simulink model "v2012_DynStab"  (Simulink 7.6)
settings: Solver=ode45  StartTime=0.0  StopTime=10.0  RelTol=1e-3
libraries: fm_lib x1
(part 1 of 4)
settings Model: Creator=davidusb  LastModifiedBy=davidusb

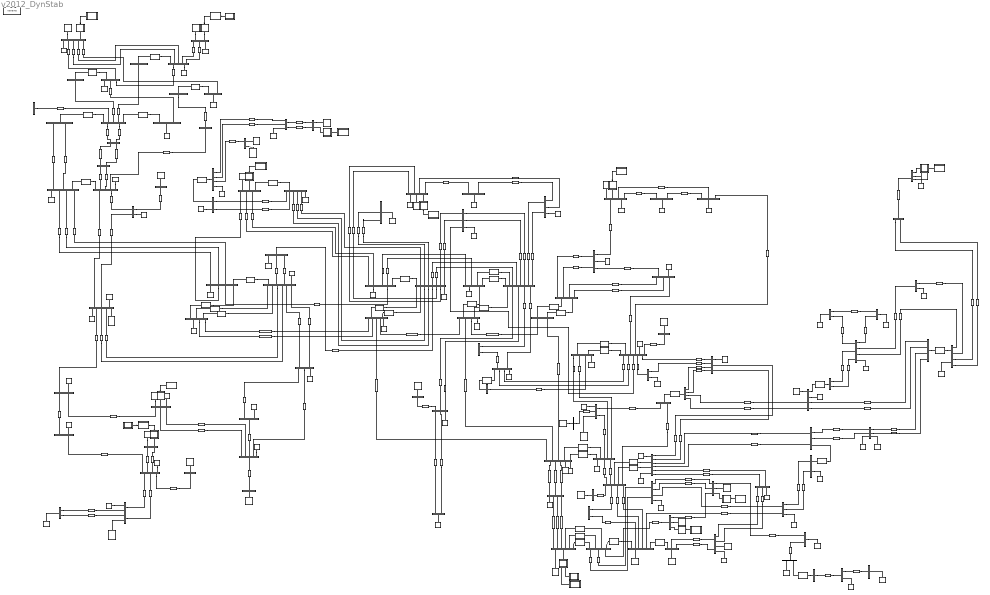
== system v2012_DynStab ==
  note: Hacia Empresas
      | Mixtas PDVSA
  note: REACTOR
      | 3x300
  note: REACTOR
      | 4x300
  note: COMP
      | ESTATICO
  note: REACTOR
      | 2x50
  note: Guri 400 kV
  note: Macagua I y III
  note: Caruachi
  note: Macagua II
  note: S/E San Geronimo 765kV
  note: S/E Malena 765kV
  note: S/E Guri 765kV
  note: Ciudad
      | Guayana
  note: Guri 230 kV
  note: Droop = ~0 ==> isochronous mode
  note: (AT adicional 150MVA 2012)
  note: 2x100MVAr
      | SHUNT CAP
  note: Puerto La Cruz
  note: Caracas
  note: Maracay
  note: S/E Sur 765kV
  note: REACTOR
      | 2x100
  note: (2da linea 2012)
  note: Valencia
  note: S/E La Horqueta 765kV
  note: S/E La Arenosa 765kV
  note: LIBRE
  note: Elaborado por: Ing. David Hernández Torres, PhD
      |
      | VERSION: 20 de Noviembre de 2012 (Simplificada, niveles de tensión: 765, 400 y 230 kV)
      | (Solo se considera una pequeña parte de la red oriental en 115kV)
      | Modelo dinámico para estudios de estabilidad
      |
      | Fuentes:
      | Elaborado siguiendo diagrama unifilar actualizado hasta el 2003 (OPSIS) y las actualizaciones
      | del sistema descritas en el Anuario Estadístico del MPPEE hasta el año 2010 y en los
      | informe anuales OPSIS 2005-2008. Finalmente el modelo 2012 se obtiene luego de actualización
      | del modelo 2010 bajo las premisas descritas en los archivos pronostico_demanda_electrica.xls y
      | Datos SEN.xls
      |
      | (Es necesaria la instalación del toolbox PSAT, el esquema se elaboró con Simulink
      | y la version 7.11 R2010b de Matlab, se puede ejecutar el archivo de datos .m desde Octave y la
      | version de PSAT correspondiente)
  note: SISTEMA ELECTRICO NACIONAL
  note: COMP
      | ESTATICO
  note: REACTOR
      | 2x50
  note: REACTOR
      | 1x300
  note: REACTOR
      | 2x25
  note: Cumana
  note: REACTOR
      | 1x50
  note: Isla de Margarita
  note: REACTOR
      | 2x25
  note: Brasil
  note: REACTOR
      | 2x50
  note: TAP=1.1
  note: Termozulia
      | Rafael Urdaneta
  note: CAPACITOR
      | 1x108
  note: REACTOR
      | 1x50
  note: REACTOR
      | 4x50
  note: SERIES
      | CAPACITOR
      | COMP
      | 3x50 OHM
  note: Maracaibo
  note: HACIA COLOMBIA
  note: REACTOR
      | 1x300
  note: REACTOR
      | 4x50
  note: LIBRE
  note: LIBRE
  note: S/E Yaracuy 765kV
  note: Barquisimeto
  note: Merida
  note: San Cristobal
  note: Colombia
  note: REACTOR
      | 2x20
  note: Peninsula de Paraguaná
  note: (2da linea 2012)
  AVR1 : Subsystem  Tag=PSATblock  Description=Controls  mask(Exc){p2q=2, p3q=inf, p4q=0, p5q=200, p6q=0.02, p7q=0.01, p8q=1.0, p9q=1, p10q=0.7, p11q=0.001, p12_13q=[0.0006  0.9], in=0}
      mask prompts: p2q "Automatic Voltage Regulator Type"; p3q "Maximum Regulator Voltage [p.u.]"; p4q "Minimum Regulator Voltage [p.u.]"; p5q "Amplifier Gain Ka [p.u./p.u.]"; p6q "Amplifier Time Constant Ta [s]"; p7q "Stabilizer Gain Kf [p.u./p.u.]"; p8q "Stabilizer Time Tf [s]"; p9q "Integral deviation Ke [p.u./p.u.]"; p10q "Time Constant of the Field Circuit Td [s]"; p11q "Time Delay of the Measurement System Tr [s]"; p12_13q "Coefficient of the Ceiling Function (A B)"; in "Number of input signals"
      mask help: This block defines an Automatic Voltage Regulator.
      mask init:
      | fm_inout
      | [x,y] = fm_draw('R');
      mask Help:
      | This block defines an Automatic Voltage Regulator.
      | There are three kind of regulators:
      | 
      | Type 1:
      | 
      |      IEEE Model 1
      | 
      | Type 2:
      | 
      |      IEEE Model 2
      | 
      | Type 3:
      | 
      |      IEEE Model 3
      mask StyleString: popup(1|2|3),edit,edit,edit,edit,edit,edit,edit,edit,edit,edit,popup(0|1|2|3)
      mask CallbackString: fm_block|||||||||||
      mask Display:
      | plot([-1.8 4.1 4.1 -1.8 -1.8],[-1.5 -1.5 1.5 1.5 -1.5])
      | color('red')
      | plot([-1.3 -0.5],[-1 1],[-0.5 0.3],[1 -1],[-0.9 -0.1],[0.0 0.0])
      | plot(2.8+1.3*x,2*y,1.5+[-1.3 -0.5],[1 -1],1.5+[-0.5 0.3],[-1 1])
  AVR10 : Subsystem  Tag=PSATblock  Description=Controls  mask(Exc){p2q=2, p3q=7.3, p4q=-7.3, p5q=400, p6q=0.02, p7q=0.03, p8q=1.0, p9q=1, p10q=0.253, p11q=0.001, p12_13q=[0.0006  0.9], in=0}
      mask prompts: p2q "Automatic Voltage Regulator Type"; p3q "Maximum Regulator Voltage [p.u.]"; p4q "Minimum Regulator Voltage [p.u.]"; p5q "Amplifier Gain Ka [p.u./p.u.]"; p6q "Amplifier Time Constant Ta [s]"; p7q "Stabilizer Gain Kf [p.u./p.u.]"; p8q "Stabilizer Time Tf [s]"; p9q "Integral deviation Ke [p.u./p.u.]"; p10q "Time Constant of the Field Circuit Td [s]"; p11q "Time Delay of the Measurement System Tr [s]"; p12_13q "Coefficient of the Ceiling Function (A B)"; in "Number of input signals"
      mask help: This block defines an Automatic Voltage Regulator.
      mask init:
      | fm_inout
      | [x,y] = fm_draw('R');
      mask Help:
      | This block defines an Automatic Voltage Regulator.
      | There are three kind of regulators:
      | 
      | Type 1:
      | 
      |      IEEE Model 1
      | 
      | Type 2:
      | 
      |      IEEE Model 2
      | 
      | Type 3:
      | 
      |      IEEE Model 3
      mask StyleString: popup(1|2|3),edit,edit,edit,edit,edit,edit,edit,edit,edit,edit,popup(0|1|2|3)
      mask CallbackString: fm_block|||||||||||
      mask Display:
      | plot([-1.8 4.1 4.1 -1.8 -1.8],[-1.5 -1.5 1.5 1.5 -1.5])
      | color('red')
      | plot([-1.3 -0.5],[-1 1],[-0.5 0.3],[1 -1],[-0.9 -0.1],[0.0 0.0])
      | plot(2.8+1.3*x,2*y,1.5+[-1.3 -0.5],[1 -1],1.5+[-0.5 0.3],[-1 1])
  AVR11 : Subsystem  Tag=PSATblock  Description=Controls  mask(Exc){p2q=2, p3q=7.3, p4q=-7.3, p5q=400, p6q=0.02, p7q=0.03, p8q=1.0, p9q=1, p10q=0.253, p11q=0.001, p12_13q=[0.0006  0.9], in=0}
      mask prompts: p2q "Automatic Voltage Regulator Type"; p3q "Maximum Regulator Voltage [p.u.]"; p4q "Minimum Regulator Voltage [p.u.]"; p5q "Amplifier Gain Ka [p.u./p.u.]"; p6q "Amplifier Time Constant Ta [s]"; p7q "Stabilizer Gain Kf [p.u./p.u.]"; p8q "Stabilizer Time Tf [s]"; p9q "Integral deviation Ke [p.u./p.u.]"; p10q "Time Constant of the Field Circuit Td [s]"; p11q "Time Delay of the Measurement System Tr [s]"; p12_13q "Coefficient of the Ceiling Function (A B)"; in "Number of input signals"
      mask help: This block defines an Automatic Voltage Regulator.
      mask init:
      | fm_inout
      | [x,y] = fm_draw('R');
      mask Help:
      | This block defines an Automatic Voltage Regulator.
      | There are three kind of regulators:
      | 
      | Type 1:
      | 
      |      IEEE Model 1
      | 
      | Type 2:
      | 
      |      IEEE Model 2
      | 
      | Type 3:
      | 
      |      IEEE Model 3
      mask StyleString: popup(1|2|3),edit,edit,edit,edit,edit,edit,edit,edit,edit,edit,popup(0|1|2|3)
      mask CallbackString: fm_block|||||||||||
      mask Display:
      | plot([-1.8 4.1 4.1 -1.8 -1.8],[-1.5 -1.5 1.5 1.5 -1.5])
      | color('red')
      | plot([-1.3 -0.5],[-1 1],[-0.5 0.3],[1 -1],[-0.9 -0.1],[0.0 0.0])
      | plot(2.8+1.3*x,2*y,1.5+[-1.3 -0.5],[1 -1],1.5+[-0.5 0.3],[-1 1])
  AVR12 : Subsystem  Tag=PSATblock  Description=Controls  mask(Exc){p2q=2, p3q=50, p4q=-7.3, p5q=400, p6q=0.02, p7q=0.03, p8q=1.0, p9q=1, p10q=0.253, p11q=0.001, p12_13q=[0.0006  0.9], in=0}
      mask prompts: p2q "Automatic Voltage Regulator Type"; p3q "Maximum Regulator Voltage [p.u.]"; p4q "Minimum Regulator Voltage [p.u.]"; p5q "Amplifier Gain Ka [p.u./p.u.]"; p6q "Amplifier Time Constant Ta [s]"; p7q "Stabilizer Gain Kf [p.u./p.u.]"; p8q "Stabilizer Time Tf [s]"; p9q "Integral deviation Ke [p.u./p.u.]"; p10q "Time Constant of the Field Circuit Td [s]"; p11q "Time Delay of the Measurement System Tr [s]"; p12_13q "Coefficient of the Ceiling Function (A B)"; in "Number of input signals"
      mask help: This block defines an Automatic Voltage Regulator.
      mask init:
      | fm_inout
      | [x,y] = fm_draw('R');
      mask Help:
      | This block defines an Automatic Voltage Regulator.
      | There are three kind of regulators:
      | 
      | Type 1:
      | 
      |      IEEE Model 1
      | 
      | Type 2:
      | 
      |      IEEE Model 2
      | 
      | Type 3:
      | 
      |      IEEE Model 3
      mask StyleString: popup(1|2|3),edit,edit,edit,edit,edit,edit,edit,edit,edit,edit,popup(0|1|2|3)
      mask CallbackString: fm_block|||||||||||
      mask Display:
      | plot([-1.8 4.1 4.1 -1.8 -1.8],[-1.5 -1.5 1.5 1.5 -1.5])
      | color('red')
      | plot([-1.3 -0.5],[-1 1],[-0.5 0.3],[1 -1],[-0.9 -0.1],[0.0 0.0])
      | plot(2.8+1.3*x,2*y,1.5+[-1.3 -0.5],[1 -1],1.5+[-0.5 0.3],[-1 1])
  AVR13 : Subsystem  Tag=PSATblock  Description=Controls  mask(Exc){p2q=2, p3q=50, p4q=-3.84, p5q=200, p6q=0.395, p7q=0.0635, p8q=1.0, p9q=1, p10q=0.001, p11q=0.001, p12_13q=[0.0006  0.9], in=0}
      mask prompts: p2q "Automatic Voltage Regulator Type"; p3q "Maximum Regulator Voltage [p.u.]"; p4q "Minimum Regulator Voltage [p.u.]"; p5q "Amplifier Gain Ka [p.u./p.u.]"; p6q "Amplifier Time Constant Ta [s]"; p7q "Stabilizer Gain Kf [p.u./p.u.]"; p8q "Stabilizer Time Tf [s]"; p9q "Integral deviation Ke [p.u./p.u.]"; p10q "Time Constant of the Field Circuit Td [s]"; p11q "Time Delay of the Measurement System Tr [s]"; p12_13q "Coefficient of the Ceiling Function (A B)"; in "Number of input signals"
      mask help: This block defines an Automatic Voltage Regulator.
      mask init:
      | fm_inout
      | [x,y] = fm_draw('R');
      mask Help:
      | This block defines an Automatic Voltage Regulator.
      | There are three kind of regulators:
      | 
      | Type 1:
      | 
      |      IEEE Model 1
      | 
      | Type 2:
      | 
      |      IEEE Model 2
      | 
      | Type 3:
      | 
      |      IEEE Model 3
      mask StyleString: popup(1|2|3),edit,edit,edit,edit,edit,edit,edit,edit,edit,edit,popup(0|1|2|3)
      mask CallbackString: fm_block|||||||||||
      mask Display:
      | plot([-1.8 4.1 4.1 -1.8 -1.8],[-1.5 -1.5 1.5 1.5 -1.5])
      | color('red')
      | plot([-1.3 -0.5],[-1 1],[-0.5 0.3],[1 -1],[-0.9 -0.1],[0.0 0.0])
      | plot(2.8+1.3*x,2*y,1.5+[-1.3 -0.5],[1 -1],1.5+[-0.5 0.3],[-1 1])
  AVR2 : Subsystem  Tag=PSATblock  Description=Controls  mask(Exc){p2q=2, p3q=7.3, p4q=-7.3, p5q=400, p6q=0.02, p7q=0.03, p8q=1.0, p9q=1, p10q=0.253, p11q=0.001, p12_13q=[0.0006  0.9], in=0}
      mask prompts: p2q "Automatic Voltage Regulator Type"; p3q "Maximum Regulator Voltage [p.u.]"; p4q "Minimum Regulator Voltage [p.u.]"; p5q "Amplifier Gain Ka [p.u./p.u.]"; p6q "Amplifier Time Constant Ta [s]"; p7q "Stabilizer Gain Kf [p.u./p.u.]"; p8q "Stabilizer Time Tf [s]"; p9q "Integral deviation Ke [p.u./p.u.]"; p10q "Time Constant of the Field Circuit Td [s]"; p11q "Time Delay of the Measurement System Tr [s]"; p12_13q "Coefficient of the Ceiling Function (A B)"; in "Number of input signals"
      mask help: This block defines an Automatic Voltage Regulator.
      mask init:
      | fm_inout
      | [x,y] = fm_draw('R');
      mask Help:
      | This block defines an Automatic Voltage Regulator.
      | There are three kind of regulators:
      | 
      | Type 1:
      | 
      |      IEEE Model 1
      | 
      | Type 2:
      | 
      |      IEEE Model 2
      | 
      | Type 3:
      | 
      |      IEEE Model 3
      mask StyleString: popup(1|2|3),edit,edit,edit,edit,edit,edit,edit,edit,edit,edit,popup(0|1|2|3)
      mask CallbackString: fm_block|||||||||||
      mask Display:
      | plot([-1.8 4.1 4.1 -1.8 -1.8],[-1.5 -1.5 1.5 1.5 -1.5])
      | color('red')
      | plot([-1.3 -0.5],[-1 1],[-0.5 0.3],[1 -1],[-0.9 -0.1],[0.0 0.0])
      | plot(2.8+1.3*x,2*y,1.5+[-1.3 -0.5],[1 -1],1.5+[-0.5 0.3],[-1 1])
  AVR3 : Subsystem  Tag=PSATblock  Description=Controls  mask(Exc){p2q=2, p3q=1, p4q=-1, p5q=50, p6q=0.06, p7q=0.07, p8q=1.0, p9q=-0.0393, p10q=0.44, p11q=0.001, p12_13q=[0.0006  0.9], in=1}
      mask prompts: p2q "Automatic Voltage Regulator Type"; p3q "Maximum Regulator Voltage [p.u.]"; p4q "Minimum Regulator Voltage [p.u.]"; p5q "Amplifier Gain Ka [p.u./p.u.]"; p6q "Amplifier Time Constant Ta [s]"; p7q "Stabilizer Gain Kf [p.u./p.u.]"; p8q "Stabilizer Time Tf [s]"; p9q "Integral deviation Ke [p.u./p.u.]"; p10q "Time Constant of the Field Circuit Td [s]"; p11q "Time Delay of the Measurement System Tr [s]"; p12_13q "Coefficient of the Ceiling Function (A B)"; in "Number of input signals"
      mask help: This block defines an Automatic Voltage Regulator.
      mask init:
      | fm_inout
      | [x,y] = fm_draw('R');
      mask Help:
      | This block defines an Automatic Voltage Regulator.
      | There are three kind of regulators:
      | 
      | Type 1:
      | 
      |      IEEE Model 1
      | 
      | Type 2:
      | 
      |      IEEE Model 2
      | 
      | Type 3:
      | 
      |      IEEE Model 3
      mask StyleString: popup(1|2|3),edit,edit,edit,edit,edit,edit,edit,edit,edit,edit,popup(0|1|2|3)
      mask CallbackString: fm_block|||||||||||
      mask Display:
      | plot([-1.8 4.1 4.1 -1.8 -1.8],[-1.5 -1.5 1.5 1.5 -1.5])
      | color('red')
      | plot([-1.3 -0.5],[-1 1],[-0.5 0.3],[1 -1],[-0.9 -0.1],[0.0 0.0])
      | plot(2.8+1.3*x,2*y,1.5+[-1.3 -0.5],[1 -1],1.5+[-0.5 0.3],[-1 1])
  AVR4 : Subsystem  Tag=PSATblock  Description=Controls  mask(Exc){p2q=2, p3q=10, p4q=-3.84, p5q=200, p6q=0.395, p7q=0.0635, p8q=1.0, p9q=1, p10q=0.001, p11q=0.001, p12_13q=[0.0006  0.9], in=0}
      mask prompts: p2q "Automatic Voltage Regulator Type"; p3q "Maximum Regulator Voltage [p.u.]"; p4q "Minimum Regulator Voltage [p.u.]"; p5q "Amplifier Gain Ka [p.u./p.u.]"; p6q "Amplifier Time Constant Ta [s]"; p7q "Stabilizer Gain Kf [p.u./p.u.]"; p8q "Stabilizer Time Tf [s]"; p9q "Integral deviation Ke [p.u./p.u.]"; p10q "Time Constant of the Field Circuit Td [s]"; p11q "Time Delay of the Measurement System Tr [s]"; p12_13q "Coefficient of the Ceiling Function (A B)"; in "Number of input signals"
      mask help: This block defines an Automatic Voltage Regulator.
      mask init:
      | fm_inout
      | [x,y] = fm_draw('R');
      mask Help:
      | This block defines an Automatic Voltage Regulator.
      | There are three kind of regulators:
      | 
      | Type 1:
      | 
      |      IEEE Model 1
      | 
      | Type 2:
      | 
      |      IEEE Model 2
      | 
      | Type 3:
      | 
      |      IEEE Model 3
      mask StyleString: popup(1|2|3),edit,edit,edit,edit,edit,edit,edit,edit,edit,edit,popup(0|1|2|3)
      mask CallbackString: fm_block|||||||||||
      mask Display:
      | plot([-1.8 4.1 4.1 -1.8 -1.8],[-1.5 -1.5 1.5 1.5 -1.5])
      | color('red')
      | plot([-1.3 -0.5],[-1 1],[-0.5 0.3],[1 -1],[-0.9 -0.1],[0.0 0.0])
      | plot(2.8+1.3*x,2*y,1.5+[-1.3 -0.5],[1 -1],1.5+[-0.5 0.3],[-1 1])
  AVR5 : Subsystem  Tag=PSATblock  Description=Controls  mask(Exc){p2q=2, p3q=10, p4q=-1, p5q=50, p6q=0.06, p7q=0.0648, p8q=1.0, p9q=-0.08, p10q=0.405, p11q=0.001, p12_13q=[0.0006  0.9], in=0}
      mask prompts: p2q "Automatic Voltage Regulator Type"; p3q "Maximum Regulator Voltage [p.u.]"; p4q "Minimum Regulator Voltage [p.u.]"; p5q "Amplifier Gain Ka [p.u./p.u.]"; p6q "Amplifier Time Constant Ta [s]"; p7q "Stabilizer Gain Kf [p.u./p.u.]"; p8q "Stabilizer Time Tf [s]"; p9q "Integral deviation Ke [p.u./p.u.]"; p10q "Time Constant of the Field Circuit Td [s]"; p11q "Time Delay of the Measurement System Tr [s]"; p12_13q "Coefficient of the Ceiling Function (A B)"; in "Number of input signals"
      mask help: This block defines an Automatic Voltage Regulator.
      mask init:
      | fm_inout
      | [x,y] = fm_draw('R');
      mask Help:
      | This block defines an Automatic Voltage Regulator.
      | There are three kind of regulators:
      | 
      | Type 1:
      | 
      |      IEEE Model 1
      | 
      | Type 2:
      | 
      |      IEEE Model 2
      | 
      | Type 3:
      | 
      |      IEEE Model 3
      mask StyleString: popup(1|2|3),edit,edit,edit,edit,edit,edit,edit,edit,edit,edit,popup(0|1|2|3)
      mask CallbackString: fm_block|||||||||||
      mask Display:
      | plot([-1.8 4.1 4.1 -1.8 -1.8],[-1.5 -1.5 1.5 1.5 -1.5])
      | color('red')
      | plot([-1.3 -0.5],[-1 1],[-0.5 0.3],[1 -1],[-0.9 -0.1],[0.0 0.0])
      | plot(2.8+1.3*x,2*y,1.5+[-1.3 -0.5],[1 -1],1.5+[-0.5 0.3],[-1 1])
  AVR6 : Subsystem  Tag=PSATblock  Description=Controls  mask(Exc){p2q=2, p3q=inf, p4q=-1, p5q=50, p6q=0.06, p7q=0.0648, p8q=1.0, p9q=-0.08, p10q=0.405, p11q=0.001, p12_13q=[0.0006  0.9], in=0}
      mask prompts: p2q "Automatic Voltage Regulator Type"; p3q "Maximum Regulator Voltage [p.u.]"; p4q "Minimum Regulator Voltage [p.u.]"; p5q "Amplifier Gain Ka [p.u./p.u.]"; p6q "Amplifier Time Constant Ta [s]"; p7q "Stabilizer Gain Kf [p.u./p.u.]"; p8q "Stabilizer Time Tf [s]"; p9q "Integral deviation Ke [p.u./p.u.]"; p10q "Time Constant of the Field Circuit Td [s]"; p11q "Time Delay of the Measurement System Tr [s]"; p12_13q "Coefficient of the Ceiling Function (A B)"; in "Number of input signals"
      mask help: This block defines an Automatic Voltage Regulator.
      mask init:
      | fm_inout
      | [x,y] = fm_draw('R');
      mask Help:
      | This block defines an Automatic Voltage Regulator.
      | There are three kind of regulators:
      | 
      | Type 1:
      | 
      |      IEEE Model 1
      | 
      | Type 2:
      | 
      |      IEEE Model 2
      | 
      | Type 3:
      | 
      |      IEEE Model 3
      mask StyleString: popup(1|2|3),edit,edit,edit,edit,edit,edit,edit,edit,edit,edit,popup(0|1|2|3)
      mask CallbackString: fm_block|||||||||||
      mask Display:
      | plot([-1.8 4.1 4.1 -1.8 -1.8],[-1.5 -1.5 1.5 1.5 -1.5])
      | color('red')
      | plot([-1.3 -0.5],[-1 1],[-0.5 0.3],[1 -1],[-0.9 -0.1],[0.0 0.0])
      | plot(2.8+1.3*x,2*y,1.5+[-1.3 -0.5],[1 -1],1.5+[-0.5 0.3],[-1 1])
  AVR7 : Subsystem  Tag=PSATblock  Description=Controls  mask(Exc){p2q=2, p3q=1, p4q=-1, p5q=50, p6q=0.06, p7q=0.0648, p8q=1.0, p9q=-0.08, p10q=0.405, p11q=0.001, p12_13q=[0.0006  0.9], in=0}
      mask prompts: p2q "Automatic Voltage Regulator Type"; p3q "Maximum Regulator Voltage [p.u.]"; p4q "Minimum Regulator Voltage [p.u.]"; p5q "Amplifier Gain Ka [p.u./p.u.]"; p6q "Amplifier Time Constant Ta [s]"; p7q "Stabilizer Gain Kf [p.u./p.u.]"; p8q "Stabilizer Time Tf [s]"; p9q "Integral deviation Ke [p.u./p.u.]"; p10q "Time Constant of the Field Circuit Td [s]"; p11q "Time Delay of the Measurement System Tr [s]"; p12_13q "Coefficient of the Ceiling Function (A B)"; in "Number of input signals"
      mask help: This block defines an Automatic Voltage Regulator.
      mask init:
      | fm_inout
      | [x,y] = fm_draw('R');
      mask Help:
      | This block defines an Automatic Voltage Regulator.
      | There are three kind of regulators:
      | 
      | Type 1:
      | 
      |      IEEE Model 1
      | 
      | Type 2:
      | 
      |      IEEE Model 2
      | 
      | Type 3:
      | 
      |      IEEE Model 3
      mask StyleString: popup(1|2|3),edit,edit,edit,edit,edit,edit,edit,edit,edit,edit,popup(0|1|2|3)
      mask CallbackString: fm_block|||||||||||
      mask Display:
      | plot([-1.8 4.1 4.1 -1.8 -1.8],[-1.5 -1.5 1.5 1.5 -1.5])
      | color('red')
      | plot([-1.3 -0.5],[-1 1],[-0.5 0.3],[1 -1],[-0.9 -0.1],[0.0 0.0])
      | plot(2.8+1.3*x,2*y,1.5+[-1.3 -0.5],[1 -1],1.5+[-0.5 0.3],[-1 1])
  AVR8 : Subsystem  Tag=PSATblock  Description=Controls  mask(Exc){p2q=2, p3q=1, p4q=-1, p5q=50, p6q=0.06, p7q=0.0648, p8q=1.0, p9q=-0.08, p10q=0.405, p11q=0.001, p12_13q=[0.0006  0.9], in=1}
      mask prompts: p2q "Automatic Voltage Regulator Type"; p3q "Maximum Regulator Voltage [p.u.]"; p4q "Minimum Regulator Voltage [p.u.]"; p5q "Amplifier Gain Ka [p.u./p.u.]"; p6q "Amplifier Time Constant Ta [s]"; p7q "Stabilizer Gain Kf [p.u./p.u.]"; p8q "Stabilizer Time Tf [s]"; p9q "Integral deviation Ke [p.u./p.u.]"; p10q "Time Constant of the Field Circuit Td [s]"; p11q "Time Delay of the Measurement System Tr [s]"; p12_13q "Coefficient of the Ceiling Function (A B)"; in "Number of input signals"
      mask help: This block defines an Automatic Voltage Regulator.
      mask init:
      | fm_inout
      | [x,y] = fm_draw('R');
      mask Help:
      | This block defines an Automatic Voltage Regulator.
      | There are three kind of regulators:
      | 
      | Type 1:
      | 
      |      IEEE Model 1
      | 
      | Type 2:
      | 
      |      IEEE Model 2
      | 
      | Type 3:
      | 
      |      IEEE Model 3
      mask StyleString: popup(1|2|3),edit,edit,edit,edit,edit,edit,edit,edit,edit,edit,popup(0|1|2|3)
      mask CallbackString: fm_block|||||||||||
      mask Display:
      | plot([-1.8 4.1 4.1 -1.8 -1.8],[-1.5 -1.5 1.5 1.5 -1.5])
      | color('red')
      | plot([-1.3 -0.5],[-1 1],[-0.5 0.3],[1 -1],[-0.9 -0.1],[0.0 0.0])
      | plot(2.8+1.3*x,2*y,1.5+[-1.3 -0.5],[1 -1],1.5+[-0.5 0.3],[-1 1])
  Acarigua II 230kV : PMComponent  Tag=PSATblock  Description=Connection  PhysicalDomain=psatdomain  LeftPortType=p1  RightPortType=p1  LConnTagsString=__newl0|__newl1  RConnTagsString=__newr0|__newr1|__newr2  mask(Bus){in=2, out=3, p2q=230, p3_4q=[0.96856    -0.61292], p5q=1, p6q=1}
      mask prompts: in "Number of inputs:"; out "Number of outputs:"; p2q "Voltage Rating [kV]"; p3_4q "Voltage initial guess [p.u.  rad]"; p5q "Area number"; p6q "Region number"
      mask help: Bus block.
      mask init:
      | fm_inout
      settings: AttributesFormatString="|V| =  0.9862 p.u.\\n<V  = -0.3303 rad"
      mask CallbackString: ||||fm_block|
      mask Display: plot([0 1 1 0 0],[0 0 1 1 0])
  Aragua 230kV : PMComponent  Tag=PSATblock  Description=Connection  PhysicalDomain=psatdomain  LeftPortType=p1  RightPortType=p1  LConnTagsString=__newl0|__newl1|__newl2  RConnTagsString=__newr0|__newr1|__newr2  mask(Bus){in=3, out=3, p2q=230, p3_4q=[0.953    -0.54917], p5q=1, p6q=1}
      mask prompts: in "Number of inputs:"; out "Number of outputs:"; p2q "Voltage Rating [kV]"; p3_4q "Voltage initial guess [p.u.  rad]"; p5q "Area number"; p6q "Region number"
      mask help: Bus block.
      mask init:
      | fm_inout
      settings: AttributesFormatString="|V| =  0.9768 p.u.\\n<V  = -0.3545 rad"
      mask CallbackString: ||||fm_block|
      mask Display: plot([0 1 1 0 0],[0 0 1 1 0])
  Auto : PMComponent  Tag=PSATblock  Description=Power Flow  PhysicalDomain=psatdomain  LeftPortType=p1  RightPortType=p1  LConnTagsString=__newl0  RConnTagsString=__newr0  mask(Line){p3_4_5q=[1500  765 60], p7q=1.9124, p8q=0.01, p9q=0.20, p13_14_15q=[0.0  0.0  0.0], p16q=on}
      mask prompts: p3_4_5q "Power, Voltage and Frequency Ratings [MVA, kV, Hz]"; p7q "Primary and secondary voltage ratio [kV/kV]"; p8q "Resistance [p.u.]"; p9q "Reactance [p.u.]"; p13_14_15q "Imax, Pmax and Smax [p.u., p.u., p.u.]"; p16q "Connected"
      mask help: This block defines an auto-transformer.
      mask init:
      | [x,y] = fm_draw('circle');
      | [xq,yq] = fm_draw('quarter');
      mask CallbackString: |||||fm_block
      mask Display: plot(x,y,1.75*xq,yq,[-1 -1.3],[0 0],[1.75 2.05],[0 0])
  Auto1 : PMComponent  Tag=PSATblock  Description=Power Flow  PhysicalDomain=psatdomain  LeftPortType=p1  RightPortType=p1  LConnTagsString=__newl0  RConnTagsString=__newr0  mask(Line){p3_4_5q=[1500  765 60], p7q=1.9124, p8q=0.01, p9q=0.20, p13_14_15q=[0.0  0.0  0.0], p16q=on}
      mask prompts: p3_4_5q "Power, Voltage and Frequency Ratings [MVA, kV, Hz]"; p7q "Primary and secondary voltage ratio [kV/kV]"; p8q "Resistance [p.u.]"; p9q "Reactance [p.u.]"; p13_14_15q "Imax, Pmax and Smax [p.u., p.u., p.u.]"; p16q "Connected"
      mask help: This block defines an auto-transformer.
      mask init:
      | [x,y] = fm_draw('circle');
      | [xq,yq] = fm_draw('quarter');
      mask CallbackString: |||||fm_block
      mask Display: plot(x,y,1.75*xq,yq,[-1 -1.3],[0 0],[1.75 2.05],[0 0])
  Auto11 : PMComponent  Tag=PSATblock  Description=Power Flow  PhysicalDomain=psatdomain  LeftPortType=p1  RightPortType=p1  LConnTagsString=__newl0  RConnTagsString=__newr0  mask(Line){p3_4_5q=[900  400 60], p7q=1.7391, p8q=0.01, p9q=0.20, p13_14_15q=[0.0  0.0  0.0], p16q=on}
      mask prompts: p3_4_5q "Power, Voltage and Frequency Ratings [MVA, kV, Hz]"; p7q "Primary and secondary voltage ratio [kV/kV]"; p8q "Resistance [p.u.]"; p9q "Reactance [p.u.]"; p13_14_15q "Imax, Pmax and Smax [p.u., p.u., p.u.]"; p16q "Connected"
      mask help: This block defines an auto-transformer.
      mask init:
      | [x,y] = fm_draw('circle');
      | [xq,yq] = fm_draw('quarter');
      mask CallbackString: |||||fm_block
      mask Display: plot(x,y,1.75*xq,yq,[-1 -1.3],[0 0],[1.75 2.05],[0 0])
  Auto17 : PMComponent  Tag=PSATblock  Description=Power Flow  PhysicalDomain=psatdomain  LeftPortType=p1  RightPortType=p1  LConnTagsString=__newl0  RConnTagsString=__newr0  mask(Line){p3_4_5q=[450  400 60], p7q=1.7391, p8q=0.01, p9q=0.20, p13_14_15q=[0.0  0.0  0.0], p16q=on}
      mask prompts: p3_4_5q "Power, Voltage and Frequency Ratings [MVA, kV, Hz]"; p7q "Primary and secondary voltage ratio [kV/kV]"; p8q "Resistance [p.u.]"; p9q "Reactance [p.u.]"; p13_14_15q "Imax, Pmax and Smax [p.u., p.u., p.u.]"; p16q "Connected"
      mask help: This block defines an auto-transformer.
      mask init:
      | [x,y] = fm_draw('circle');
      | [xq,yq] = fm_draw('quarter');
      mask CallbackString: |||||fm_block
      mask Display: plot(x,y,1.75*xq,yq,[-1 -1.3],[0 0],[1.75 2.05],[0 0])
  Auto19 : PMComponent  Tag=PSATblock  Description=Power Flow  PhysicalDomain=psatdomain  LeftPortType=p1  RightPortType=p1  LConnTagsString=__newl0  RConnTagsString=__newr0  mask(Line){p3_4_5q=[450  400 60], p7q=1.7391, p8q=0.01, p9q=0.20, p13_14_15q=[0.0  0.0  0.0], p16q=on}
      mask prompts: p3_4_5q "Power, Voltage and Frequency Ratings [MVA, kV, Hz]"; p7q "Primary and secondary voltage ratio [kV/kV]"; p8q "Resistance [p.u.]"; p9q "Reactance [p.u.]"; p13_14_15q "Imax, Pmax and Smax [p.u., p.u., p.u.]"; p16q "Connected"
      mask help: This block defines an auto-transformer.
      mask init:
      | [x,y] = fm_draw('circle');
      | [xq,yq] = fm_draw('quarter');
      mask CallbackString: |||||fm_block
      mask Display: plot(x,y,1.75*xq,yq,[-1 -1.3],[0 0],[1.75 2.05],[0 0])
  Auto2 : PMComponent  Tag=PSATblock  Description=Power Flow  PhysicalDomain=psatdomain  LeftPortType=p1  RightPortType=p1  LConnTagsString=__newl0  RConnTagsString=__newr0  mask(Line){p3_4_5q=[1500  765 60], p7q=1.9124, p8q=0.01, p9q=0.20, p13_14_15q=[0.0  0.0  0.0], p16q=on}
      mask prompts: p3_4_5q "Power, Voltage and Frequency Ratings [MVA, kV, Hz]"; p7q "Primary and secondary voltage ratio [kV/kV]"; p8q "Resistance [p.u.]"; p9q "Reactance [p.u.]"; p13_14_15q "Imax, Pmax and Smax [p.u., p.u., p.u.]"; p16q "Connected"
      mask help: This block defines an auto-transformer.
      mask init:
      | [x,y] = fm_draw('circle');
      | [xq,yq] = fm_draw('quarter');
      mask CallbackString: |||||fm_block
      mask Display: plot(x,y,1.75*xq,yq,[-1 -1.3],[0 0],[1.75 2.05],[0 0])
  Auto20 : PMComponent  Tag=PSATblock  Description=Power Flow  PhysicalDomain=psatdomain  LeftPortType=p1  RightPortType=p1  LConnTagsString=__newl0  RConnTagsString=__newr0  mask(Line){p3_4_5q=[450  400 60], p7q=1.7391, p8q=0.01, p9q=0.20, p13_14_15q=[0.0  0.0  0.0], p16q=on}
      mask prompts: p3_4_5q "Power, Voltage and Frequency Ratings [MVA, kV, Hz]"; p7q "Primary and secondary voltage ratio [kV/kV]"; p8q "Resistance [p.u.]"; p9q "Reactance [p.u.]"; p13_14_15q "Imax, Pmax and Smax [p.u., p.u., p.u.]"; p16q "Connected"
      mask help: This block defines an auto-transformer.
      mask init:
      | [x,y] = fm_draw('circle');
      | [xq,yq] = fm_draw('quarter');
      mask CallbackString: |||||fm_block
      mask Display: plot(x,y,1.75*xq,yq,[-1 -1.3],[0 0],[1.75 2.05],[0 0])
  Auto21 : PMComponent  Tag=PSATblock  Description=Power Flow  PhysicalDomain=psatdomain  LeftPortType=p1  RightPortType=p1  LConnTagsString=__newl0  RConnTagsString=__newr0  mask(Line){p3_4_5q=[1000  765 60], p7q=3.3256, p8q=0.01, p9q=0.20, p13_14_15q=[0.0  0.0  0.0], p16q=on}
      mask prompts: p3_4_5q "Power, Voltage and Frequency Ratings [MVA, kV, Hz]"; p7q "Primary and secondary voltage ratio [kV/kV]"; p8q "Resistance [p.u.]"; p9q "Reactance [p.u.]"; p13_14_15q "Imax, Pmax and Smax [p.u., p.u., p.u.]"; p16q "Connected"
      mask help: This block defines an auto-transformer.
      mask init:
      | [x,y] = fm_draw('circle');
      | [xq,yq] = fm_draw('quarter');
      mask CallbackString: |||||fm_block
      mask Display: plot(x,y,1.75*xq,yq,[-1 -1.3],[0 0],[1.75 2.05],[0 0])
  Auto22 : PMComponent  Tag=PSATblock  Description=Power Flow  PhysicalDomain=psatdomain  LeftPortType=p1  RightPortType=p1  LConnTagsString=__newl0  RConnTagsString=__newr0  mask(Line){p3_4_5q=[1000  765 60], p7q=3.3256, p8q=0.01, p9q=0.20, p13_14_15q=[0.0  0.0  0.0], p16q=on}
      mask prompts: p3_4_5q "Power, Voltage and Frequency Ratings [MVA, kV, Hz]"; p7q "Primary and secondary voltage ratio [kV/kV]"; p8q "Resistance [p.u.]"; p9q "Reactance [p.u.]"; p13_14_15q "Imax, Pmax and Smax [p.u., p.u., p.u.]"; p16q "Connected"
      mask help: This block defines an auto-transformer.
      mask init:
      | [x,y] = fm_draw('circle');
      | [xq,yq] = fm_draw('quarter');
      mask CallbackString: |||||fm_block
      mask Display: plot(x,y,1.75*xq,yq,[-1 -1.3],[0 0],[1.75 2.05],[0 0])
  Auto23 : PMComponent  Tag=PSATblock  Description=Power Flow  PhysicalDomain=psatdomain  LeftPortType=p1  RightPortType=p1  LConnTagsString=__newl0  RConnTagsString=__newr0  mask(Line){p3_4_5q=[1500  765 60], p7q=1.9124, p8q=0.01, p9q=0.20, p13_14_15q=[0.0  0.0  0.0], p16q=on}
      mask prompts: p3_4_5q "Power, Voltage and Frequency Ratings [MVA, kV, Hz]"; p7q "Primary and secondary voltage ratio [kV/kV]"; p8q "Resistance [p.u.]"; p9q "Reactance [p.u.]"; p13_14_15q "Imax, Pmax and Smax [p.u., p.u., p.u.]"; p16q "Connected"
      mask help: This block defines an auto-transformer.
      mask init:
      | [x,y] = fm_draw('circle');
      | [xq,yq] = fm_draw('quarter');
      mask CallbackString: |||||fm_block
      mask Display: plot(x,y,1.75*xq,yq,[-1 -1.3],[0 0],[1.75 2.05],[0 0])
  Auto24 : PMComponent  Tag=PSATblock  Description=Power Flow  PhysicalDomain=psatdomain  LeftPortType=p1  RightPortType=p1  LConnTagsString=__newl0  RConnTagsString=__newr0  mask(Line){p3_4_5q=[450 400 60], p7q=1.7391, p8q=0.01, p9q=0.20, p13_14_15q=[0.0  0.0  0.0], p16q=on}
      mask prompts: p3_4_5q "Power, Voltage and Frequency Ratings [MVA, kV, Hz]"; p7q "Primary and secondary voltage ratio [kV/kV]"; p8q "Resistance [p.u.]"; p9q "Reactance [p.u.]"; p13_14_15q "Imax, Pmax and Smax [p.u., p.u., p.u.]"; p16q "Connected"
      mask help: This block defines an auto-transformer.
      mask init:
      | [x,y] = fm_draw('circle');
      | [xq,yq] = fm_draw('quarter');
      mask CallbackString: |||||fm_block
      mask Display: plot(x,y,1.75*xq,yq,[-1 -1.3],[0 0],[1.75 2.05],[0 0])
  Auto25 : PMComponent  Tag=PSATblock  Description=Power Flow  PhysicalDomain=psatdomain  LeftPortType=p1  RightPortType=p1  LConnTagsString=__newl0  RConnTagsString=__newr0  mask(Line){p3_4_5q=[450 400 60], p7q=1.7391, p8q=0.01, p9q=0.20, p13_14_15q=[0.0  0.0  0.0], p16q=on}
      mask prompts: p3_4_5q "Power, Voltage and Frequency Ratings [MVA, kV, Hz]"; p7q "Primary and secondary voltage ratio [kV/kV]"; p8q "Resistance [p.u.]"; p9q "Reactance [p.u.]"; p13_14_15q "Imax, Pmax and Smax [p.u., p.u., p.u.]"; p16q "Connected"
      mask help: This block defines an auto-transformer.
      mask init:
      | [x,y] = fm_draw('circle');
      | [xq,yq] = fm_draw('quarter');
      mask CallbackString: |||||fm_block
      mask Display: plot(x,y,1.75*xq,yq,[-1 -1.3],[0 0],[1.75 2.05],[0 0])
  Auto26 : PMComponent  Tag=PSATblock  Description=Power Flow  PhysicalDomain=psatdomain  LeftPortType=p1  RightPortType=p1  LConnTagsString=__newl0  RConnTagsString=__newr0  mask(Line){p3_4_5q=[1000 765 60], p7q=3.3256, p8q=0.01, p9q=0.20, p13_14_15q=[0.0  0.0  0.0], p16q=on}
      mask prompts: p3_4_5q "Power, Voltage and Frequency Ratings [MVA, kV, Hz]"; p7q "Primary and secondary voltage ratio [kV/kV]"; p8q "Resistance [p.u.]"; p9q "Reactance [p.u.]"; p13_14_15q "Imax, Pmax and Smax [p.u., p.u., p.u.]"; p16q "Connected"
      mask help: This block defines an auto-transformer.
      mask init:
      | [x,y] = fm_draw('circle');
      | [xq,yq] = fm_draw('quarter');
      mask CallbackString: |||||fm_block
      mask Display: plot(x,y,1.75*xq,yq,[-1 -1.3],[0 0],[1.75 2.05],[0 0])
  Auto27 : PMComponent  Tag=PSATblock  Description=Power Flow  PhysicalDomain=psatdomain  LeftPortType=p1  RightPortType=p1  LConnTagsString=__newl0  RConnTagsString=__newr0  mask(Line){p3_4_5q=[1000 765 60], p7q=3.3256, p8q=0.01, p9q=0.20, p13_14_15q=[0.0  0.0  0.0], p16q=on}
      mask prompts: p3_4_5q "Power, Voltage and Frequency Ratings [MVA, kV, Hz]"; p7q "Primary and secondary voltage ratio [kV/kV]"; p8q "Resistance [p.u.]"; p9q "Reactance [p.u.]"; p13_14_15q "Imax, Pmax and Smax [p.u., p.u., p.u.]"; p16q "Connected"
      mask help: This block defines an auto-transformer.
      mask init:
      | [x,y] = fm_draw('circle');
      | [xq,yq] = fm_draw('quarter');
      mask CallbackString: |||||fm_block
      mask Display: plot(x,y,1.75*xq,yq,[-1 -1.3],[0 0],[1.75 2.05],[0 0])
  Auto28 : PMComponent  Tag=PSATblock  Description=Power Flow  PhysicalDomain=psatdomain  LeftPortType=p1  RightPortType=p1  LConnTagsString=__newl0  RConnTagsString=__newr0  mask(Line){p3_4_5q=[1000 765 60], p7q=3.3256, p8q=0.01, p9q=0.20, p13_14_15q=[0.0  0.0  0.0], p16q=on}
      mask prompts: p3_4_5q "Power, Voltage and Frequency Ratings [MVA, kV, Hz]"; p7q "Primary and secondary voltage ratio [kV/kV]"; p8q "Resistance [p.u.]"; p9q "Reactance [p.u.]"; p13_14_15q "Imax, Pmax and Smax [p.u., p.u., p.u.]"; p16q "Connected"
      mask help: This block defines an auto-transformer.
      mask init:
      | [x,y] = fm_draw('circle');
      | [xq,yq] = fm_draw('quarter');
      mask CallbackString: |||||fm_block
      mask Display: plot(x,y,1.75*xq,yq,[-1 -1.3],[0 0],[1.75 2.05],[0 0])
  Auto29 : PMComponent  Tag=PSATblock  Description=Power Flow  PhysicalDomain=psatdomain  LeftPortType=p1  RightPortType=p1  LConnTagsString=__newl0  RConnTagsString=__newr0  mask(Line){p3_4_5q=[900 400 60], p7q=1.7391, p8q=0.01, p9q=0.20, p13_14_15q=[0.0  0.0  0.0], p16q=on}
      mask prompts: p3_4_5q "Power, Voltage and Frequency Ratings [MVA, kV, Hz]"; p7q "Primary and secondary voltage ratio [kV/kV]"; p8q "Resistance [p.u.]"; p9q "Reactance [p.u.]"; p13_14_15q "Imax, Pmax and Smax [p.u., p.u., p.u.]"; p16q "Connected"
      mask help: This block defines an auto-transformer.
      mask init:
      | [x,y] = fm_draw('circle');
      | [xq,yq] = fm_draw('quarter');
      mask CallbackString: |||||fm_block
      mask Display: plot(x,y,1.75*xq,yq,[-1 -1.3],[0 0],[1.75 2.05],[0 0])
  Auto3 : PMComponent  Tag=PSATblock  Description=Power Flow  PhysicalDomain=psatdomain  LeftPortType=p1  RightPortType=p1  LConnTagsString=__newl0  RConnTagsString=__newr0  mask(Line){p3_4_5q=[450  400 60], p7q=1.7391, p8q=0.01, p9q=0.20, p13_14_15q=[0.0  0.0  0.0], p16q=on}
      mask prompts: p3_4_5q "Power, Voltage and Frequency Ratings [MVA, kV, Hz]"; p7q "Primary and secondary voltage ratio [kV/kV]"; p8q "Resistance [p.u.]"; p9q "Reactance [p.u.]"; p13_14_15q "Imax, Pmax and Smax [p.u., p.u., p.u.]"; p16q "Connected"
      mask help: This block defines an auto-transformer.
      mask init:
      | [x,y] = fm_draw('circle');
      | [xq,yq] = fm_draw('quarter');
      mask CallbackString: |||||fm_block
      mask Display: plot(x,y,1.75*xq,yq,[-1 -1.3],[0 0],[1.75 2.05],[0 0])
  Auto37 : PMComponent  Tag=PSATblock  Description=Power Flow  PhysicalDomain=psatdomain  LeftPortType=p1  RightPortType=p1  LConnTagsString=__newl0  RConnTagsString=__newr0  mask(Line){p3_4_5q=[450 400 60], p7q=1.7391, p8q=0.01, p9q=0.20, p13_14_15q=[0.0  0.0  0.0], p16q=on}
      mask prompts: p3_4_5q "Power, Voltage and Frequency Ratings [MVA, kV, Hz]"; p7q "Primary and secondary voltage ratio [kV/kV]"; p8q "Resistance [p.u.]"; p9q "Reactance [p.u.]"; p13_14_15q "Imax, Pmax and Smax [p.u., p.u., p.u.]"; p16q "Connected"
      mask help: This block defines an auto-transformer.
      mask init:
      | [x,y] = fm_draw('circle');
      | [xq,yq] = fm_draw('quarter');
      mask CallbackString: |||||fm_block
      mask Display: plot(x,y,1.75*xq,yq,[-1 -1.3],[0 0],[1.75 2.05],[0 0])
  Auto38 : PMComponent  Tag=PSATblock  Description=Power Flow  PhysicalDomain=psatdomain  LeftPortType=p1  RightPortType=p1  LConnTagsString=__newl0  RConnTagsString=__newr0  mask(Line){p3_4_5q=[1500  765 60], p7q=1.9124, p8q=0.01, p9q=0.20, p13_14_15q=[0.0  0.0  0.0], p16q=on}
      mask prompts: p3_4_5q "Power, Voltage and Frequency Ratings [MVA, kV, Hz]"; p7q "Primary and secondary voltage ratio [kV/kV]"; p8q "Resistance [p.u.]"; p9q "Reactance [p.u.]"; p13_14_15q "Imax, Pmax and Smax [p.u., p.u., p.u.]"; p16q "Connected"
      mask help: This block defines an auto-transformer.
      mask init:
      | [x,y] = fm_draw('circle');
      | [xq,yq] = fm_draw('quarter');
      mask CallbackString: |||||fm_block
      mask Display: plot(x,y,1.75*xq,yq,[-1 -1.3],[0 0],[1.75 2.05],[0 0])
  Auto39 : PMComponent  Tag=PSATblock  Description=Power Flow  PhysicalDomain=psatdomain  LeftPortType=p1  RightPortType=p1  LConnTagsString=__newl0  RConnTagsString=__newr0  mask(Line){p3_4_5q=[1000 765 60], p7q=3.3256, p8q=0.01, p9q=0.20, p13_14_15q=[0.0  0.0  0.0], p16q=on}
      mask prompts: p3_4_5q "Power, Voltage and Frequency Ratings [MVA, kV, Hz]"; p7q "Primary and secondary voltage ratio [kV/kV]"; p8q "Resistance [p.u.]"; p9q "Reactance [p.u.]"; p13_14_15q "Imax, Pmax and Smax [p.u., p.u., p.u.]"; p16q "Connected"
      mask help: This block defines an auto-transformer.
      mask init:
      | [x,y] = fm_draw('circle');
      | [xq,yq] = fm_draw('quarter');
      mask CallbackString: |||||fm_block
      mask Display: plot(x,y,1.75*xq,yq,[-1 -1.3],[0 0],[1.75 2.05],[0 0])
  Auto4 : PMComponent  Tag=PSATblock  Description=Power Flow  PhysicalDomain=psatdomain  LeftPortType=p1  RightPortType=p1  LConnTagsString=__newl0  RConnTagsString=__newr0  mask(Line){p3_4_5q=[1500  765 60], p7q=1.9124, p8q=0.01, p9q=0.20, p13_14_15q=[0.0  0.0  0.0], p16q=on}
      mask prompts: p3_4_5q "Power, Voltage and Frequency Ratings [MVA, kV, Hz]"; p7q "Primary and secondary voltage ratio [kV/kV]"; p8q "Resistance [p.u.]"; p9q "Reactance [p.u.]"; p13_14_15q "Imax, Pmax and Smax [p.u., p.u., p.u.]"; p16q "Connected"
      mask help: This block defines an auto-transformer.
      mask init:
      | [x,y] = fm_draw('circle');
      | [xq,yq] = fm_draw('quarter');
      mask CallbackString: |||||fm_block
      mask Display: plot(x,y,1.75*xq,yq,[-1 -1.3],[0 0],[1.75 2.05],[0 0])
  Auto40 : PMComponent  Tag=PSATblock  Description=Power Flow  PhysicalDomain=psatdomain  LeftPortType=p1  RightPortType=p1  LConnTagsString=__newl0  RConnTagsString=__newr0  mask(Line){p3_4_5q=[900 400 60], p7q=1.7391, p8q=0.01, p9q=0.20, p13_14_15q=[0.0  0.0  0.0], p16q=on}
      mask prompts: p3_4_5q "Power, Voltage and Frequency Ratings [MVA, kV, Hz]"; p7q "Primary and secondary voltage ratio [kV/kV]"; p8q "Resistance [p.u.]"; p9q "Reactance [p.u.]"; p13_14_15q "Imax, Pmax and Smax [p.u., p.u., p.u.]"; p16q "Connected"
      mask help: This block defines an auto-transformer.
      mask init:
      | [x,y] = fm_draw('circle');
      | [xq,yq] = fm_draw('quarter');
      mask CallbackString: |||||fm_block
      mask Display: plot(x,y,1.75*xq,yq,[-1 -1.3],[0 0],[1.75 2.05],[0 0])
  Auto49 : PMComponent  Tag=PSATblock  Description=Power Flow  PhysicalDomain=psatdomain  LeftPortType=p1  RightPortType=p1  LConnTagsString=__newl0  RConnTagsString=__newr0  mask(Line){p3_4_5q=[1350 400 60], p7q=1.7391, p8q=0.01, p9q=0.20, p13_14_15q=[0.0  0.0  0.0], p16q=on}
      mask prompts: p3_4_5q "Power, Voltage and Frequency Ratings [MVA, kV, Hz]"; p7q "Primary and secondary voltage ratio [kV/kV]"; p8q "Resistance [p.u.]"; p9q "Reactance [p.u.]"; p13_14_15q "Imax, Pmax and Smax [p.u., p.u., p.u.]"; p16q "Connected"
      mask help: This block defines an auto-transformer.
      mask init:
      | [x,y] = fm_draw('circle');
      | [xq,yq] = fm_draw('quarter');
      mask CallbackString: |||||fm_block
      mask Display: plot(x,y,1.75*xq,yq,[-1 -1.3],[0 0],[1.75 2.05],[0 0])
  Auto5 : PMComponent  Tag=PSATblock  Description=Power Flow  PhysicalDomain=psatdomain  LeftPortType=p1  RightPortType=p1  LConnTagsString=__newl0  RConnTagsString=__newr0  mask(Line){p3_4_5q=[1500  765 60], p7q=1.9124, p8q=0.01, p9q=0.20, p13_14_15q=[0.0  0.0  0.0], p16q=on}
      mask prompts: p3_4_5q "Power, Voltage and Frequency Ratings [MVA, kV, Hz]"; p7q "Primary and secondary voltage ratio [kV/kV]"; p8q "Resistance [p.u.]"; p9q "Reactance [p.u.]"; p13_14_15q "Imax, Pmax and Smax [p.u., p.u., p.u.]"; p16q "Connected"
      mask help: This block defines an auto-transformer.
      mask init:
      | [x,y] = fm_draw('circle');
      | [xq,yq] = fm_draw('quarter');
      mask CallbackString: |||||fm_block
      mask Display: plot(x,y,1.75*xq,yq,[-1 -1.3],[0 0],[1.75 2.05],[0 0])
  Auto50 : PMComponent  Tag=PSATblock  Description=Power Flow  PhysicalDomain=psatdomain  LeftPortType=p1  RightPortType=p1  LConnTagsString=__newl0  RConnTagsString=__newr0  mask(Line){p3_4_5q=[300  230 60], p7q=2, p8q=0.01, p9q=0.20, p13_14_15q=[0.0  0.0  0.0], p16q=on}
      mask prompts: p3_4_5q "Power, Voltage and Frequency Ratings [MVA, kV, Hz]"; p7q "Primary and secondary voltage ratio [kV/kV]"; p8q "Resistance [p.u.]"; p9q "Reactance [p.u.]"; p13_14_15q "Imax, Pmax and Smax [p.u., p.u., p.u.]"; p16q "Connected"
      mask help: This block defines an auto-transformer.
      mask init:
      | [x,y] = fm_draw('circle');
      | [xq,yq] = fm_draw('quarter');
      mask CallbackString: |||||fm_block
      mask Display: plot(x,y,1.75*xq,yq,[-1 -1.3],[0 0],[1.75 2.05],[0 0])
  Auto56 : PMComponent  Tag=PSATblock  Description=Power Flow  PhysicalDomain=psatdomain  LeftPortType=p1  RightPortType=p1  LConnTagsString=__newl0  RConnTagsString=__newr0  mask(Line){p3_4_5q=[450 400 60], p7q=1.7391, p8q=0.01, p9q=0.20, p13_14_15q=[0.0  0.0  0.0], p16q=on}
      mask prompts: p3_4_5q "Power, Voltage and Frequency Ratings [MVA, kV, Hz]"; p7q "Primary and secondary voltage ratio [kV/kV]"; p8q "Resistance [p.u.]"; p9q "Reactance [p.u.]"; p13_14_15q "Imax, Pmax and Smax [p.u., p.u., p.u.]"; p16q "Connected"
      mask help: This block defines an auto-transformer.
      mask init:
      | [x,y] = fm_draw('circle');
      | [xq,yq] = fm_draw('quarter');
      mask CallbackString: |||||fm_block
      mask Display: plot(x,y,1.75*xq,yq,[-1 -1.3],[0 0],[1.75 2.05],[0 0])
  Auto57 : PMComponent  Tag=PSATblock  Description=Power Flow  PhysicalDomain=psatdomain  LeftPortType=p1  RightPortType=p1  LConnTagsString=__newl0  RConnTagsString=__newr0  mask(Line){p3_4_5q=[333 230 60], p7q=1.6666, p8q=0.01, p9q=0.20, p13_14_15q=[0.0  0.0  0.0], p16q=on}
      mask prompts: p3_4_5q "Power, Voltage and Frequency Ratings [MVA, kV, Hz]"; p7q "Primary and secondary voltage ratio [kV/kV]"; p8q "Resistance [p.u.]"; p9q "Reactance [p.u.]"; p13_14_15q "Imax, Pmax and Smax [p.u., p.u., p.u.]"; p16q "Connected"
      mask help: This block defines an auto-transformer.
      mask init:
      | [x,y] = fm_draw('circle');
      | [xq,yq] = fm_draw('quarter');
      mask CallbackString: |||||fm_block
      mask Display: plot(x,y,1.75*xq,yq,[-1 -1.3],[0 0],[1.75 2.05],[0 0])
  Auto58 : PMComponent  Tag=PSATblock  Description=Power Flow  PhysicalDomain=psatdomain  LeftPortType=p1  RightPortType=p1  LConnTagsString=__newl0  RConnTagsString=__newr0  mask(Line){p3_4_5q=[333 230 60], p7q=1.6666, p8q=0.01, p9q=0.20, p13_14_15q=[0.0  0.0  0.0], p16q=on}
      mask prompts: p3_4_5q "Power, Voltage and Frequency Ratings [MVA, kV, Hz]"; p7q "Primary and secondary voltage ratio [kV/kV]"; p8q "Resistance [p.u.]"; p9q "Reactance [p.u.]"; p13_14_15q "Imax, Pmax and Smax [p.u., p.u., p.u.]"; p16q "Connected"
      mask help: This block defines an auto-transformer.
      mask init:
      | [x,y] = fm_draw('circle');
      | [xq,yq] = fm_draw('quarter');
      mask CallbackString: |||||fm_block
      mask Display: plot(x,y,1.75*xq,yq,[-1 -1.3],[0 0],[1.75 2.05],[0 0])
  Auto59 : PMComponent  Tag=PSATblock  Description=Power Flow  PhysicalDomain=psatdomain  LeftPortType=p1  RightPortType=p1  LConnTagsString=__newl0  RConnTagsString=__newr0  mask(Line){p3_4_5q=[333 230 60], p7q=1.6666, p8q=0.01, p9q=0.20, p13_14_15q=[0.0  0.0  0.0], p16q=on}
      mask prompts: p3_4_5q "Power, Voltage and Frequency Ratings [MVA, kV, Hz]"; p7q "Primary and secondary voltage ratio [kV/kV]"; p8q "Resistance [p.u.]"; p9q "Reactance [p.u.]"; p13_14_15q "Imax, Pmax and Smax [p.u., p.u., p.u.]"; p16q "Connected"
      mask help: This block defines an auto-transformer.
      mask init:
      | [x,y] = fm_draw('circle');
      | [xq,yq] = fm_draw('quarter');
      mask CallbackString: |||||fm_block
      mask Display: plot(x,y,1.75*xq,yq,[-1 -1.3],[0 0],[1.75 2.05],[0 0])
  Auto6 : PMComponent  Tag=PSATblock  Description=Power Flow  PhysicalDomain=psatdomain  LeftPortType=p1  RightPortType=p1  LConnTagsString=__newl0  RConnTagsString=__newr0  mask(Line){p3_4_5q=[450  400 60], p7q=1.7391, p8q=0.01, p9q=0.20, p13_14_15q=[0.0  0.0  0.0], p16q=on}
      mask prompts: p3_4_5q "Power, Voltage and Frequency Ratings [MVA, kV, Hz]"; p7q "Primary and secondary voltage ratio [kV/kV]"; p8q "Resistance [p.u.]"; p9q "Reactance [p.u.]"; p13_14_15q "Imax, Pmax and Smax [p.u., p.u., p.u.]"; p16q "Connected"
      mask help: This block defines an auto-transformer.
      mask init:
      | [x,y] = fm_draw('circle');
      | [xq,yq] = fm_draw('quarter');
      mask CallbackString: |||||fm_block
      mask Display: plot(x,y,1.75*xq,yq,[-1 -1.3],[0 0],[1.75 2.05],[0 0])
  Auto60 : PMComponent  Tag=PSATblock  Description=Power Flow  PhysicalDomain=psatdomain  LeftPortType=p1  RightPortType=p1  LConnTagsString=__newl0  RConnTagsString=__newr0  mask(Line){p3_4_5q=[333 230 60], p7q=1.6666, p8q=0.01, p9q=0.20, p13_14_15q=[0.0  0.0  0.0], p16q=on}
      mask prompts: p3_4_5q "Power, Voltage and Frequency Ratings [MVA, kV, Hz]"; p7q "Primary and secondary voltage ratio [kV/kV]"; p8q "Resistance [p.u.]"; p9q "Reactance [p.u.]"; p13_14_15q "Imax, Pmax and Smax [p.u., p.u., p.u.]"; p16q "Connected"
      mask help: This block defines an auto-transformer.
      mask init:
      | [x,y] = fm_draw('circle');
      | [xq,yq] = fm_draw('quarter');
      mask CallbackString: |||||fm_block
      mask Display: plot(x,y,1.75*xq,yq,[-1 -1.3],[0 0],[1.75 2.05],[0 0])
  Auto61 : PMComponent  Tag=PSATblock  Description=Power Flow  PhysicalDomain=psatdomain  LeftPortType=p1  RightPortType=p1  LConnTagsString=__newl0  RConnTagsString=__newr0  mask(Line){p3_4_5q=[1000  400 60], p7q=1, p8q=0.01, p9q=0.20, p13_14_15q=[0.0  0.0  0.0], p16q=on}
      mask prompts: p3_4_5q "Power, Voltage and Frequency Ratings [MVA, kV, Hz]"; p7q "Primary and secondary voltage ratio [kV/kV]"; p8q "Resistance [p.u.]"; p9q "Reactance [p.u.]"; p13_14_15q "Imax, Pmax and Smax [p.u., p.u., p.u.]"; p16q "Connected"
      mask help: This block defines an auto-transformer.
      mask init:
      | [x,y] = fm_draw('circle');
      | [xq,yq] = fm_draw('quarter');
      mask CallbackString: |||||fm_block
      mask Display: plot(x,y,1.75*xq,yq,[-1 -1.3],[0 0],[1.75 2.05],[0 0])
  Auto66 : PMComponent  Tag=PSATblock  Description=Power Flow  PhysicalDomain=psatdomain  LeftPortType=p1  RightPortType=p1  LConnTagsString=__newl0  RConnTagsString=__newr0  mask(Line){p3_4_5q=[300  400 60], p7q=1.1*400/230, p8q=0.01, p9q=0.20, p13_14_15q=[0.0  0.0  0.0], p16q=on}
      mask prompts: p3_4_5q "Power, Voltage and Frequency Ratings [MVA, kV, Hz]"; p7q "Primary and secondary voltage ratio [kV/kV]"; p8q "Resistance [p.u.]"; p9q "Reactance [p.u.]"; p13_14_15q "Imax, Pmax and Smax [p.u., p.u., p.u.]"; p16q "Connected"
      mask help: This block defines an auto-transformer.
      mask init:
      | [x,y] = fm_draw('circle');
      | [xq,yq] = fm_draw('quarter');
      mask CallbackString: |||||fm_block
      mask Display: plot(x,y,1.75*xq,yq,[-1 -1.3],[0 0],[1.75 2.05],[0 0])
  Auto7 : PMComponent  Tag=PSATblock  Description=Power Flow  PhysicalDomain=psatdomain  LeftPortType=p1  RightPortType=p1  LConnTagsString=__newl0  RConnTagsString=__newr0  mask(Line){p3_4_5q=[450  400 60], p7q=1.7391, p8q=0.01, p9q=0.20, p13_14_15q=[0.0  0.0  0.0], p16q=on}
      mask prompts: p3_4_5q "Power, Voltage and Frequency Ratings [MVA, kV, Hz]"; p7q "Primary and secondary voltage ratio [kV/kV]"; p8q "Resistance [p.u.]"; p9q "Reactance [p.u.]"; p13_14_15q "Imax, Pmax and Smax [p.u., p.u., p.u.]"; p16q "Connected"
      mask help: This block defines an auto-transformer.
      mask init:
      | [x,y] = fm_draw('circle');
      | [xq,yq] = fm_draw('quarter');
      mask CallbackString: |||||fm_block
      mask Display: plot(x,y,1.75*xq,yq,[-1 -1.3],[0 0],[1.75 2.05],[0 0])
  Auto72 : PMComponent  Tag=PSATblock  Description=Power Flow  PhysicalDomain=psatdomain  LeftPortType=p1  RightPortType=p1  LConnTagsString=__newl0  RConnTagsString=__newr0  mask(Line){p3_4_5q=[1000 765 60], p7q=3.3256, p8q=0.01, p9q=0.20, p13_14_15q=[0.0  0.0  0.0], p16q=on}
      mask prompts: p3_4_5q "Power, Voltage and Frequency Ratings [MVA, kV, Hz]"; p7q "Primary and secondary voltage ratio [kV/kV]"; p8q "Resistance [p.u.]"; p9q "Reactance [p.u.]"; p13_14_15q "Imax, Pmax and Smax [p.u., p.u., p.u.]"; p16q "Connected"
      mask help: This block defines an auto-transformer.
      mask init:
      | [x,y] = fm_draw('circle');
      | [xq,yq] = fm_draw('quarter');
      mask CallbackString: |||||fm_block
      mask Display: plot(x,y,1.75*xq,yq,[-1 -1.3],[0 0],[1.75 2.05],[0 0])
  Auto73 : PMComponent  Tag=PSATblock  Description=Power Flow  PhysicalDomain=psatdomain  LeftPortType=p1  RightPortType=p1  LConnTagsString=__newl0  RConnTagsString=__newr0  mask(Line){p3_4_5q=[600 400 60], p7q=1.7391, p8q=0.01, p9q=0.20, p13_14_15q=[0.0  0.0  0.0], p16q=on}
      mask prompts: p3_4_5q "Power, Voltage and Frequency Ratings [MVA, kV, Hz]"; p7q "Primary and secondary voltage ratio [kV/kV]"; p8q "Resistance [p.u.]"; p9q "Reactance [p.u.]"; p13_14_15q "Imax, Pmax and Smax [p.u., p.u., p.u.]"; p16q "Connected"
      mask help: This block defines an auto-transformer.
      mask init:
      | [x,y] = fm_draw('circle');
      | [xq,yq] = fm_draw('quarter');
      mask CallbackString: |||||fm_block
      mask Display: plot(x,y,1.75*xq,yq,[-1 -1.3],[0 0],[1.75 2.05],[0 0])
  Auto8 : PMComponent  Tag=PSATblock  Description=Power Flow  PhysicalDomain=psatdomain  LeftPortType=p1  RightPortType=p1  LConnTagsString=__newl0  RConnTagsString=__newr0  mask(Line){p3_4_5q=[300  230 60], p7q=2, p8q=0.01, p9q=0.20, p13_14_15q=[0.0  0.0  0.0], p16q=on}
      mask prompts: p3_4_5q "Power, Voltage and Frequency Ratings [MVA, kV, Hz]"; p7q "Primary and secondary voltage ratio [kV/kV]"; p8q "Resistance [p.u.]"; p9q "Reactance [p.u.]"; p13_14_15q "Imax, Pmax and Smax [p.u., p.u., p.u.]"; p16q "Connected"
      mask help: This block defines an auto-transformer.
      mask init:
      | [x,y] = fm_draw('circle');
      | [xq,yq] = fm_draw('quarter');
      mask CallbackString: |||||fm_block
      mask Display: plot(x,y,1.75*xq,yq,[-1 -1.3],[0 0],[1.75 2.05],[0 0])
  Auto9 : PMComponent  Tag=PSATblock  Description=Power Flow  PhysicalDomain=psatdomain  LeftPortType=p1  RightPortType=p1  LConnTagsString=__newl0  RConnTagsString=__newr0  mask(Line){p3_4_5q=[450  230 60], p7q=2, p8q=0.01, p9q=0.20, p13_14_15q=[0.0  0.0  0.0], p16q=on}
      mask prompts: p3_4_5q "Power, Voltage and Frequency Ratings [MVA, kV, Hz]"; p7q "Primary and secondary voltage ratio [kV/kV]"; p8q "Resistance [p.u.]"; p9q "Reactance [p.u.]"; p13_14_15q "Imax, Pmax and Smax [p.u., p.u., p.u.]"; p16q "Connected"
      mask help: This block defines an auto-transformer.
      mask init:
      | [x,y] = fm_draw('circle');
      | [xq,yq] = fm_draw('quarter');
      mask CallbackString: |||||fm_block
      mask Display: plot(x,y,1.75*xq,yq,[-1 -1.3],[0 0],[1.75 2.05],[0 0])
  Barbacoa I 230kV : PMComponent  Tag=PSATblock  Description=Connection  PhysicalDomain=psatdomain  LeftPortType=p1  RightPortType=p1  LConnTagsString=__newl0|__newl1|__newl2  RConnTagsString=__newr0|__newr1|__newr2|__newr3  mask(Bus){in=3, out=4, p2q=230, p3_4q=[1.0002     -0.2833], p5q=1, p6q=1}
      mask prompts: in "Number of inputs:"; out "Number of outputs:"; p2q "Voltage Rating [kV]"; p3_4q "Voltage initial guess [p.u.  rad]"; p5q "Area number"; p6q "Region number"
      mask help: Bus block.
      mask init:
      | fm_inout
      settings: AttributesFormatString="|V| =  0.9965 p.u.\\n<V  = -0.0349 rad"
      mask CallbackString: ||||fm_block|
      mask Display: plot([0 1 1 0 0],[0 0 1 1 0])
  Barbacoa II 230kV : PMComponent  Tag=PSATblock  Description=Connection  PhysicalDomain=psatdomain  LeftPortType=p1  RightPortType=p1  LConnTagsString=__newl0|__newl1|__newl2|__newl3  RConnTagsString=__newr0  mask(Bus){in=4, out=1, p2q=230, p3_4q=[1.008    -0.27165], p5q=1, p6q=1}
      mask prompts: in "Number of inputs:"; out "Number of outputs:"; p2q "Voltage Rating [kV]"; p3_4q "Voltage initial guess [p.u.  rad]"; p5q "Area number"; p6q "Region number"
      mask help: Bus block.
      mask init:
      | fm_inout
      settings: AttributesFormatString="|V| =  1.0043 p.u.\\n<V  = -0.0161 rad"
      mask CallbackString: ||||fm_block|
      mask Display: plot([0 1 1 0 0],[0 0 1 1 0])
  Barbacoa II 400kV : PMComponent  Tag=PSATblock  Description=Connection  PhysicalDomain=psatdomain  LeftPortType=p1  RightPortType=p1  LConnTagsString=__newl0|__newl1  RConnTagsString=__newr0  mask(Bus){in=2, out=1, p2q=400, p3_4q=[1.0265    -0.25382], p5q=1, p6q=1}
      mask prompts: in "Number of inputs:"; out "Number of outputs:"; p2q "Voltage Rating [kV]"; p3_4q "Voltage initial guess [p.u.  rad]"; p5q "Area number"; p6q "Region number"
      mask help: Bus block.
      mask init:
      | fm_inout
      settings: AttributesFormatString="|V| =  1.0216 p.u.\\n<V  = -0.0491 rad"
      mask CallbackString: ||||fm_block|
      mask Display: plot([0 1 1 0 0],[0 0 1 1 0])
  Barinas IV 230kV : PMComponent  Tag=PSATblock  Description=Connection  PhysicalDomain=psatdomain  LeftPortType=p1  RightPortType=p1  LConnTagsString=__newl0|__newl1|__newl2|__newl3|__newl4  RConnTagsString=__newr0  mask(Bus){in=5, out=1, p2q=230, p3_4q=[1.0576    -0.61106], p5q=1, p6q=1}
      mask prompts: in "Number of inputs:"; out "Number of outputs:"; p2q "Voltage Rating [kV]"; p3_4q "Voltage initial guess [p.u.  rad]"; p5q "Area number"; p6q "Region number"
      mask help: Bus block.
      mask init:
      | fm_inout
      settings: AttributesFormatString="|V| =  1.0488 p.u.\\n<V  = -0.2151 rad"
      mask CallbackString: ||||fm_block|
      mask Display: plot([0 1 1 0 0],[0 0 1 1 0])
  Boa Vista (Brasil) : PMComponent  Tag=PSATblock  Description=Connection  PhysicalDomain=psatdomain  LeftPortType=p1  RightPortType=p1  LConnTagsString=__newl0  RConnTagsString=__newr0  mask(Bus){in=1, out=1, p2q=230, p3_4q=[0.96771    -0.42846], p5q=1, p6q=1}
      mask prompts: in "Number of inputs:"; out "Number of outputs:"; p2q "Voltage Rating [kV]"; p3_4q "Voltage initial guess [p.u.  rad]"; p5q "Area number"; p6q "Region number"
      mask help: Bus block.
      mask init:
      | fm_inout
      settings: AttributesFormatString="|V| =  0.9331 p.u.\\n<V  = -0.4524 rad"
      mask CallbackString: ||||fm_block|
      mask Display: plot([0 1 1 0 0],[0 0 1 1 0])
  Boyaca 230kV : PMComponent  Tag=PSATblock  Description=Connection  PhysicalDomain=psatdomain  LeftPortType=p1  RightPortType=p1  LConnTagsString=__newl0|__newl1  RConnTagsString=__newr0  mask(Bus){in=2, out=1, p2q=230, p3_4q=[0.99306    -0.51836], p5q=1, p6q=1}
      mask prompts: in "Number of inputs:"; out "Number of outputs:"; p2q "Voltage Rating [kV]"; p3_4q "Voltage initial guess [p.u.  rad]"; p5q "Area number"; p6q "Region number"
      mask help: Bus block.
      mask init:
      | fm_inout
      settings: AttributesFormatString="|V| =  1.0026 p.u.\\n<V  = -0.3409 rad"
      mask CallbackString: ||||fm_block|
      mask Display: plot([0 1 1 0 0],[0 0 1 1 0])
  Buena Vista 230kV : PMComponent  Tag=PSATblock  Description=Connection  PhysicalDomain=psatdomain  LeftPortType=p1  RightPortType=p1  LConnTagsString=__newl0|__newl1  RConnTagsString=__newr0|__newr1  mask(Bus){in=2, out=2, p2q=230, p3_4q=[1.0195    -0.72939], p5q=1, p6q=1}
      mask prompts: in "Number of inputs:"; out "Number of outputs:"; p2q "Voltage Rating [kV]"; p3_4q "Voltage initial guess [p.u.  rad]"; p5q "Area number"; p6q "Region number"
      mask help: Bus block.
      mask init:
      | fm_inout
      settings: AttributesFormatString="|V| =  0.9403 p.u.\\n<V  = -0.1577 rad"
      mask CallbackString: ||||fm_block|
      mask Display: plot([0 1 1 0 0],[0 0 1 1 0])
  Cabimas 230kV : PMComponent  Tag=PSATblock  Description=Connection  PhysicalDomain=psatdomain  LeftPortType=p1  RightPortType=p1  LConnTagsString=__newl0|__newl1  RConnTagsString=__newr0|__newr1  mask(Bus){in=2, out=2, p2q=230, p3_4q=[0.95441    -0.84457], p5q=1, p6q=1}
      mask prompts: in "Number of inputs:"; out "Number of outputs:"; p2q "Voltage Rating [kV]"; p3_4q "Voltage initial guess [p.u.  rad]"; p5q "Area number"; p6q "Region number"
      mask help: Bus block.
      mask init:
      | fm_inout
      settings: AttributesFormatString="|V| =  0.9848 p.u.\\n<V  = -0.4131 rad"
      mask CallbackString: ||||fm_block|
      mask Display: plot([0 1 1 0 0],[0 0 1 1 0])
  Cabudare 230kV : PMComponent  Tag=PSATblock  Description=Connection  PhysicalDomain=psatdomain  LeftPortType=p1  RightPortType=p1  LConnTagsString=__newl0  RConnTagsString=__newr0|__newr1|__newr2  mask(Bus){in=1, out=3, p2q=230, p3_4q=[0.92897    -0.59157], p5q=1, p6q=1}
      mask prompts: in "Number of inputs:"; out "Number of outputs:"; p2q "Voltage Rating [kV]"; p3_4q "Voltage initial guess [p.u.  rad]"; p5q "Area number"; p6q "Region number"
      mask help: Bus block.
      mask init:
      | fm_inout
      settings: AttributesFormatString="|V| =  0.9584 p.u.\\n<V  = -0.3655 rad"
      mask CallbackString: ||||fm_block|
      mask Display: plot([0 1 1 0 0],[0 0 1 1 0])
  Calabozo 230kV : PMComponent  Tag=PSATblock  Description=Connection  PhysicalDomain=psatdomain  LeftPortType=p1  RightPortType=p1  LConnTagsString=__newl0|__newl1|__newl2  RConnTagsString=__newr0|__newr1|__newr2  mask(Bus){in=3, out=3, p2q=230, p3_4q=[0.99766    -0.53707], p5q=1, p6q=1}
      mask prompts: in "Number of inputs:"; out "Number of outputs:"; p2q "Voltage Rating [kV]"; p3_4q "Voltage initial guess [p.u.  rad]"; p5q "Area number"; p6q "Region number"
      mask help: Bus block.
      mask init:
      | fm_inout
      settings: AttributesFormatString="|V| =  1.0226 p.u.\\n<V  = -0.2747 rad"
      mask CallbackString: ||||fm_block|
      mask Display: plot([0 1 1 0 0],[0 0 1 1 0])
  Cariaco : PMComponent  Tag=PSATblock  Description=Connection  PhysicalDomain=psatdomain  LeftPortType=p1  RightPortType=p1  LConnTagsString=__newl0|__newl1  RConnTagsString=__newr0  mask(Bus){in=2, out=1, p2q=115, p3_4q=[0.99722    -0.20566], p5q=1, p6q=1}
      mask prompts: in "Number of inputs:"; out "Number of outputs:"; p2q "Voltage Rating [kV]"; p3_4q "Voltage initial guess [p.u.  rad]"; p5q "Area number"; p6q "Region number"
      mask help: Bus block.
      mask init:
      | fm_inout
      settings: AttributesFormatString="|V| =  0.9486 p.u.\\n<V  =  0.1396 rad"
      mask CallbackString: ||||fm_block|
      mask Display: plot([0 1 1 0 0],[0 0 1 1 0])
  Caruachi : PMComponent  Tag=PSATblock  Description=Connection  PhysicalDomain=psatdomain  LeftPortType=p1  RightPortType=p1  LConnTagsString=__newl0|__newl1|__newl2  RConnTagsString=__newr0  mask(Bus){in=3, out=1, p2q=400, p3_4q=[1.07   -0.020149], p5q=1, p6q=1}
      mask prompts: in "Number of inputs:"; out "Number of outputs:"; p2q "Voltage Rating [kV]"; p3_4q "Voltage initial guess [p.u.  rad]"; p5q "Area number"; p6q "Region number"
      mask help: Bus block.
      mask init:
      | fm_inout
      settings: AttributesFormatString="|V| =  1.03   p.u.\\n<V  = -0.0004 rad"
      mask CallbackString: ||||fm_block|
      mask Display: plot([0 1 1 0 0],[0 0 1 1 0])
  Casanay 115kV : PMComponent  Tag=PSATblock  Description=Connection  PhysicalDomain=psatdomain  LeftPortType=p1  RightPortType=p1  LConnTagsString=__newl0|__newl1  RConnTagsString=__newr0|__newr1|__newr2|__newr3  mask(Bus){in=2, out=4, p2q=115, p3_4q=[1.0009    -0.19751], p5q=1, p6q=1}
      mask prompts: in "Number of inputs:"; out "Number of outputs:"; p2q "Voltage Rating [kV]"; p3_4q "Voltage initial guess [p.u.  rad]"; p5q "Area number"; p6q "Region number"
      mask help: Bus block.
      mask init:
      | fm_inout
      settings: AttributesFormatString="|V| =  0.9508 p.u.\\n<V  =  0.1518 rad"
      mask CallbackString: ||||fm_block|
      mask Display: plot([0 1 1 0 0],[0 0 1 1 0])
  Casanay 230kV : PMComponent  Tag=PSATblock  Description=Connection  PhysicalDomain=psatdomain  LeftPortType=p1  RightPortType=p1  LConnTagsString=__newl0  RConnTagsString=__newr0|__newr1|__newr2|__newr3  mask(Bus){in=1, out=4, p2q=230, p3_4q=[1.0178    -0.22895], p5q=1, p6q=1}
      mask prompts: in "Number of inputs:"; out "Number of outputs:"; p2q "Voltage Rating [kV]"; p3_4q "Voltage initial guess [p.u.  rad]"; p5q "Area number"; p6q "Region number"
      mask help: Bus block.
      mask init:
      | fm_inout
      settings: AttributesFormatString="|V| =  0.9818 p.u.\\n<V  =  0.0306 rad"
      mask CallbackString: ||||fm_block|
      mask Display: plot([0 1 1 0 0],[0 0 1 1 0])
  Caña de Azucar 230kV : PMComponent  Tag=PSATblock  Description=Connection  PhysicalDomain=psatdomain  LeftPortType=p1  RightPortType=p1  LConnTagsString=__newl0|__newl1  RConnTagsString=__newr0  mask(Bus){in=2, out=1, p2q=230, p3_4q=[0.94143    -0.58376], p5q=1, p6q=1}
      mask prompts: in "Number of inputs:"; out "Number of outputs:"; p2q "Voltage Rating [kV]"; p3_4q "Voltage initial guess [p.u.  rad]"; p5q "Area number"; p6q "Region number"
      mask help: Bus block.
      mask init:
      | fm_inout
      settings: AttributesFormatString="|V| =  1.007  p.u.\\n<V  = -0.4033 rad"
      mask CallbackString: ||||fm_block|
      mask Display: plot([0 1 1 0 0],[0 0 1 1 0])
  Chicopata : PMComponent  Tag=PSATblock  Description=Connection  PhysicalDomain=psatdomain  LeftPortType=p1  RightPortType=p1  LConnTagsString=__newl0|__newl1  RConnTagsString=__newr0  mask(Bus){in=2, out=1, p2q=115, p3_4q=[1.0447   -0.081846], p5q=1, p6q=1}
      mask prompts: in "Number of inputs:"; out "Number of outputs:"; p2q "Voltage Rating [kV]"; p3_4q "Voltage initial guess [p.u.  rad]"; p5q "Area number"; p6q "Region number"
      mask help: Bus block.
      mask init:
      | fm_inout
      settings: AttributesFormatString="|V| =  1.0271 p.u.\\n<V  =  0.3945 rad"
      mask CallbackString: ||||fm_block|
      mask Display: plot([0 1 1 0 0],[0 0 1 1 0])
  Ciudad Bolivar 230kV : PMComponent  Tag=PSATblock  Description=Connection  PhysicalDomain=psatdomain  LeftPortType=p1  RightPortType=p1  LConnTagsString=__newl0|__newl1  RConnTagsString=__newr0|__newr1|__newr2  mask(Bus){in=2, out=3, p2q=230, p3_4q=[1.0183    -0.23912], p5q=1, p6q=1}
      mask prompts: in "Number of inputs:"; out "Number of outputs:"; p2q "Voltage Rating [kV]"; p3_4q "Voltage initial guess [p.u.  rad]"; p5q "Area number"; p6q "Region number"
      mask help: Bus block.
      mask init:
      | fm_inout
      settings: AttributesFormatString="|V| =  0.9783 p.u.\\n<V  = -0.0806 rad"
      mask CallbackString: ||||fm_block|
      mask Display: plot([0 1 1 0 0],[0 0 1 1 0])
  Ciudad Losada 230kV : PMComponent  Tag=PSATblock  Description=Connection  PhysicalDomain=psatdomain  LeftPortType=p1  RightPortType=p1  LConnTagsString=__newl0|__newl1|__newl2|__newl3  RConnTagsString=__newr0|__newr1  mask(Bus){in=4, out=2, p2q=230, p3_4q=[0.9367    -0.47429], p5q=1, p6q=1}
      mask prompts: in "Number of inputs:"; out "Number of outputs:"; p2q "Voltage Rating [kV]"; p3_4q "Voltage initial guess [p.u.  rad]"; p5q "Area number"; p6q "Region number"
      mask help: Bus block.
      mask init:
      | fm_inout
      settings: AttributesFormatString="|V| =  1.0053 p.u.\\n<V  = -0.2677 rad"
      mask CallbackString: ||||fm_block|
      mask Display: plot([0 1 1 0 0],[0 0 1 1 0])
  Ciudad Losada 400kV : PMComponent  Tag=PSATblock  Description=Connection  PhysicalDomain=psatdomain  LeftPortType=p1  RightPortType=p1  LConnTagsString=__newl0  RConnTagsString=__newr0  mask(Bus){in=1, out=1, p2q=400, p3_4q=[0.90978    -0.37531], p5q=1, p6q=1}
      mask prompts: in "Number of inputs:"; out "Number of outputs:"; p2q "Voltage Rating [kV]"; p3_4q "Voltage initial guess [p.u.  rad]"; p5q "Area number"; p6q "Region number"
      mask help: Bus block.
      mask init:
      | fm_inout
      settings: AttributesFormatString="|V| =  1.0316 p.u.\\n<V  = -0.2085 rad"
      mask CallbackString: ||||fm_block|
      mask Display: plot([0 1 1 0 0],[0 0 1 1 0])
  Convento 230kV : PMComponent  Tag=PSATblock  Description=Connection  PhysicalDomain=psatdomain  LeftPortType=p1  RightPortType=p1  LConnTagsString=__newl0|__newl1|__newl2  RConnTagsString=__newr0  mask(Bus){in=3, out=1, p2q=230, p3_4q=[0.97044    -0.53562], p5q=1, p6q=1}
      mask prompts: in "Number of inputs:"; out "Number of outputs:"; p2q "Voltage Rating [kV]"; p3_4q "Voltage initial guess [p.u.  rad]"; p5q "Area number"; p6q "Region number"
      mask help: Bus block.
      mask init:
      | fm_inout
      settings: AttributesFormatString="|V| =  0.9875 p.u.\\n<V  = -0.3538 rad"
      mask CallbackString: ||||fm_block|
      mask Display: plot([0 1 1 0 0],[0 0 1 1 0])
  Coro II : PMComponent  Tag=PSATblock  Description=Connection  PhysicalDomain=psatdomain  LeftPortType=p1  RightPortType=p1  LConnTagsString=__newl0|__newl1  RConnTagsString=__newr0|__newr1  mask(Bus){in=2, out=2, p2q=115, p3_4q=[1.02      -0.118], p5q=1, p6q=1}
      mask prompts: in "Number of inputs:"; out "Number of outputs:"; p2q "Voltage Rating [kV]"; p3_4q "Voltage initial guess [p.u.  rad]"; p5q "Area number"; p6q "Region number"
      mask help: Bus block.
      mask init:
      | fm_inout
      settings: AttributesFormatString="|V| =  1.07   p.u.\\n<V  =  0.4841 rad"
      mask CallbackString: ||||fm_block|
      mask Display: plot([0 1 1 0 0],[0 0 1 1 0])
  Cuatricentenario 138kV : PMComponent  Tag=PSATblock  Description=Connection  PhysicalDomain=psatdomain  LeftPortType=p1  RightPortType=p1  LConnTagsString=__newl0  RConnTagsString=__newr0|__newr1  mask(Bus){in=1, out=2, p2q=138, p3_4q=[1.0046    -0.90972], p5q=1, p6q=1}
      mask prompts: in "Number of inputs:"; out "Number of outputs:"; p2q "Voltage Rating [kV]"; p3_4q "Voltage initial guess [p.u.  rad]"; p5q "Area number"; p6q "Region number"
      mask help: Bus block.
      mask init:
      | fm_inout
      settings: AttributesFormatString="|V| =  1.0004 p.u.\\n<V  = -0.3789 rad"
      mask CallbackString: ||||fm_block|
      mask Display: plot([0 1 1 0 0],[0 0 1 1 0])
  Cuatricentenario 230kV : PMComponent  Tag=PSATblock  Description=Connection  PhysicalDomain=psatdomain  LeftPortType=p1  RightPortType=p1  LConnTagsString=__newl0|__newl1|__newl2|__newl3|__newl4  RConnTagsString=__newr0|__newr1  mask(Bus){in=5, out=2, p2q=230, p3_4q=[0.99316    -0.83224], p5q=1, p6q=1}
      mask prompts: in "Number of inputs:"; out "Number of outputs:"; p2q "Voltage Rating [kV]"; p3_4q "Voltage initial guess [p.u.  rad]"; p5q "Area number"; p6q "Region number"
      mask help: Bus block.
      mask init:
      | fm_inout
      settings: AttributesFormatString="|V| =  1.0341 p.u.\\n<V  = -0.3696 rad"
      mask CallbackString: ||||fm_block|
      mask Display: plot([0 1 1 0 0],[0 0 1 1 0])
  Cuatricentenario 400kV : PMComponent  Tag=PSATblock  Description=Connection  PhysicalDomain=psatdomain  LeftPortType=p1  RightPortType=p1  LConnTagsString=__newl0  RConnTagsString=__newr0|__newr1  mask(Bus){in=1, out=2, p2q=400, p3_4q=[0.96966    -0.72924], p5q=1, p6q=1}
      mask prompts: in "Number of inputs:"; out "Number of outputs:"; p2q "Voltage Rating [kV]"; p3_4q "Voltage initial guess [p.u.  rad]"; p5q "Area number"; p6q "Region number"
      mask help: Bus block.
      mask init:
      | fm_inout
      settings: AttributesFormatString="|V| =  1.0488 p.u.\\n<V  = -0.3490 rad"
      mask CallbackString: ||||fm_block|
      mask Display: plot([0 1 1 0 0],[0 0 1 1 0])
  Cuestecita (Colombia) : PMComponent  Tag=PSATblock  Description=Connection  PhysicalDomain=psatdomain  LeftPortType=p1  RightPortType=p1  LConnTagsString=__newl0  RConnTagsString=__newr0  mask(Bus){in=1, out=1, p2q=230, p3_4q=[1.0059    -0.83355], p5q=1, p6q=1}
      mask prompts: in "Number of inputs:"; out "Number of outputs:"; p2q "Voltage Rating [kV]"; p3_4q "Voltage initial guess [p.u.  rad]"; p5q "Area number"; p6q "Region number"
      mask help: Bus block.
      mask init:
      | fm_inout
      settings: AttributesFormatString="|V| =  1.0474 p.u.\\n<V  = -0.3709 rad"
      mask CallbackString: ||||fm_block|
      mask Display: plot([0 1 1 0 0],[0 0 1 1 0])
  Cumana II : PMComponent  Tag=PSATblock  Description=Connection  PhysicalDomain=psatdomain  LeftPortType=p1  RightPortType=p1  LConnTagsString=__newl0|__newl1|__newl2  RConnTagsString=__newr0|__newr1|__newr2|__newr3  mask(Bus){in=3, out=4, p2q=115, p3_4q=[0.98444    -0.26004], p5q=1, p6q=1}
      mask prompts: in "Number of inputs:"; out "Number of outputs:"; p2q "Voltage Rating [kV]"; p3_4q "Voltage initial guess [p.u.  rad]"; p5q "Area number"; p6q "Region number"
      mask help: Bus block.
      mask init:
      | fm_inout
      settings: AttributesFormatString="|V| =  0.9568 p.u.\\n<V  =  0.0517 rad"
      mask CallbackString: ||||fm_block|
      mask Display: plot([0 1 1 0 0],[0 0 1 1 0])
  Cumana III : PMComponent  Tag=PSATblock  Description=Connection  PhysicalDomain=psatdomain  LeftPortType=p1  RightPortType=p1  LConnTagsString=__newl0|__newl1  RConnTagsString=__newr0  mask(Bus){in=2, out=1, p2q=115, p3_4q=[0.98025    -0.26446], p5q=1, p6q=1}
      mask prompts: in "Number of inputs:"; out "Number of outputs:"; p2q "Voltage Rating [kV]"; p3_4q "Voltage initial guess [p.u.  rad]"; p5q "Area number"; p6q "Region number"
      mask help: Bus block.
      mask init:
      | fm_inout
      settings: AttributesFormatString="|V| =  0.9522 p.u.\\n<V  =  0.0466 rad"
      mask CallbackString: ||||fm_block|
      mask Display: plot([0 1 1 0 0],[0 0 1 1 0])
  El Callao II 400kV : PMComponent  Tag=PSATblock  Description=Connection  PhysicalDomain=psatdomain  LeftPortType=p1  RightPortType=p1  LConnTagsString=__newl0  RConnTagsString=__newr0|__newr1  mask(Bus){in=1, out=2, p2q=400, p3_4q=[1.1192    -0.12256], p5q=1, p6q=1}
      mask prompts: in "Number of inputs:"; out "Number of outputs:"; p2q "Voltage Rating [kV]"; p3_4q "Voltage initial guess [p.u.  rad]"; p5q "Area number"; p6q "Region number"
      mask help: Bus block.
      mask init:
      | fm_inout
      settings: AttributesFormatString="|V| =  1.0717 p.u.\\n<V  = -0.1124 rad"
      mask CallbackString: ||||fm_block|
      mask Display: plot([0 1 1 0 0],[0 0 1 1 0])
  El Corozo 230kV : PMComponent  Tag=PSATblock  Description=Connection  PhysicalDomain=psatdomain  LeftPortType=p1  RightPortType=p1  LConnTagsString=__newl0|__newl1  RConnTagsString=__newr0|__newr1|__newr2|__newr3  mask(Bus){in=2, out=4, p2q=230, p3_4q=[1.0561    -0.68744], p5q=1, p6q=1}
      mask prompts: in "Number of inputs:"; out "Number of outputs:"; p2q "Voltage Rating [kV]"; p3_4q "Voltage initial guess [p.u.  rad]"; p5q "Area number"; p6q "Region number"
      mask help: Bus block.
      mask init:
      | fm_inout
      settings: AttributesFormatString="|V| =  1.0212 p.u.\\n<V  =  0.6438 rad"
      mask CallbackString: ||||fm_block|
      mask Display: plot([0 1 1 0 0],[0 0 1 1 0])
  El Indio 230kV : PMComponent  Tag=PSATblock  Description=Connection  PhysicalDomain=psatdomain  LeftPortType=p1  RightPortType=p1  LConnTagsString=__newl0|__newl1|__newl2  RConnTagsString=__newr0|__newr1|__newr2  mask(Bus){in=3, out=3, p2q=230, p3_4q=[1.0055    -0.23512], p5q=1, p6q=1}
      mask prompts: in "Number of inputs:"; out "Number of outputs:"; p2q "Voltage Rating [kV]"; p3_4q "Voltage initial guess [p.u.  rad]"; p5q "Area number"; p6q "Region number"
      mask help: Bus block.
      mask init:
      | fm_inout
      settings: AttributesFormatString="|V| =  0.9597 p.u.\\n<V  = -0.0731 rad"
      mask CallbackString: ||||fm_block|
      mask Display: plot([0 1 1 0 0],[0 0 1 1 0])
  El Rincon 138kV : PMComponent  Tag=PSATblock  Description=Connection  PhysicalDomain=psatdomain  LeftPortType=p1  RightPortType=p1  LConnTagsString=__newl0|__newl1  RConnTagsString=__newr0|__newr1|__newr2|__newr3|__newr4  mask(Bus){in=2, out=5, p2q=138, p3_4q=[1.0573    -0.90473], p5q=1, p6q=1}
      mask prompts: in "Number of inputs:"; out "Number of outputs:"; p2q "Voltage Rating [kV]"; p3_4q "Voltage initial guess [p.u.  rad]"; p5q "Area number"; p6q "Region number"
      mask help: Bus block.
      mask init:
      | fm_inout
      settings: AttributesFormatString="|V| =  1.0383 p.u.\\n<V  = -0.3054 rad"
      mask CallbackString: ||||fm_block|
      mask Display: plot([0 1 1 0 0],[0 0 1 1 0])
  El Rincon 230kV : PMComponent  Tag=PSATblock  Description=Connection  PhysicalDomain=psatdomain  LeftPortType=p1  RightPortType=p1  LConnTagsString=__newl0  RConnTagsString=__newr0  mask(Bus){in=1, out=1, p2q=230, p3_4q=[1.0067    -0.85005], p5q=1, p6q=1}
      mask prompts: in "Number of inputs:"; out "Number of outputs:"; p2q "Voltage Rating [kV]"; p3_4q "Voltage initial guess [p.u.  rad]"; p5q "Area number"; p6q "Region number"
      mask help: Bus block.
      mask init:
      | fm_inout
      settings: AttributesFormatString="|V| =  1.0355 p.u.\\n<V  = -0.3551 rad"
      mask CallbackString: ||||fm_block|
      mask Display: plot([0 1 1 0 0],[0 0 1 1 0])
  El Tablazo 230kV : PMComponent  Tag=PSATblock  Description=Connection  PhysicalDomain=psatdomain  LeftPortType=p1  RightPortType=p1  LConnTagsString=__newl0|__newl1|__newl2|__newl3|__newl4  RConnTagsString=__newr0|__newr1  mask(Bus){in=5, out=2, p2q=230, p3_4q=[0.98193    -0.81876], p5q=1, p6q=1}
      mask prompts: in "Number of inputs:"; out "Number of outputs:"; p2q "Voltage Rating [kV]"; p3_4q "Voltage initial guess [p.u.  rad]"; p5q "Area number"; p6q "Region number"
      mask help: Bus block.
      mask init:
      | fm_inout
      settings: AttributesFormatString="|V| =  1.0273 p.u.\\n<V  = -0.3801 rad"
      mask CallbackString: ||||fm_block|
      mask Display: plot([0 1 1 0 0],[0 0 1 1 0])
  El Tablazo 400kV : PMComponent  Tag=PSATblock  Description=Connection  PhysicalDomain=psatdomain  LeftPortType=p1  RightPortType=p1  LConnTagsString=__newl0|__newl1|__newl2  RConnTagsString=__newr0|__newr1|__newr2|__newr3  mask(Bus){in=3, out=4, p2q=400, p3_4q=[0.96726    -0.71909], p5q=1, p6q=1}
      mask prompts: in "Number of inputs:"; out "Number of outputs:"; p2q "Voltage Rating [kV]"; p3_4q "Voltage initial guess [p.u.  rad]"; p5q "Area number"; p6q "Region number"
      mask help: Bus block.
      mask init:
      | fm_inout
      settings: AttributesFormatString="|V| =  1.049  p.u.\\n<V  = -0.3470 rad"
      mask CallbackString: ||||fm_block|
      mask Display: plot([0 1 1 0 0],[0 0 1 1 0])
  El Tigre 230kV : PMComponent  Tag=PSATblock  Description=Connection  PhysicalDomain=psatdomain  LeftPortType=p1  RightPortType=p1  LConnTagsString=__newl0|__newl1|__newl2|__newl3|__newl4|__newl5  RConnTagsString=__newr0|__newr1|__newr2|__newr3  mask(Bus){in=6, out=4, p2q=230, p3_4q=[0.975    -0.21147], p5q=1, p6q=1}
      mask prompts: in "Number of inputs:"; out "Number of outputs:"; p2q "Voltage Rating [kV]"; p3_4q "Voltage initial guess [p.u.  rad]"; p5q "Area number"; p6q "Region number"
      mask help: Bus block.
      mask init:
      | fm_inout
      settings: AttributesFormatString="|V| =  0.9455 p.u.\\n<V  = -0.0535 rad"
      mask CallbackString: ||||fm_block|
      mask Display: plot([0 1 1 0 0],[0 0 1 1 0])
  El Tigre 400kV : PMComponent  Tag=PSATblock  Description=Connection  PhysicalDomain=psatdomain  LeftPortType=p1  RightPortType=p1  LConnTagsString=__newl0|__newl1|__newl2|__newl3|__newl4  RConnTagsString=__newr0|__newr1|__newr2|__newr3  mask(Bus){in=5, out=4, p2q=400, p3_4q=[1.0506    -0.17198], p5q=1, p6q=1}
      mask prompts: in "Number of inputs:"; out "Number of outputs:"; p2q "Voltage Rating [kV]"; p3_4q "Voltage initial guess [p.u.  rad]"; p5q "Area number"; p6q "Region number"
      mask help: Bus block.
      mask init:
      | fm_inout
      settings: AttributesFormatString="|V| =  1.0267 p.u.\\n<V  = -0.0362 rad"
      mask CallbackString: ||||fm_block|
      mask Display: plot([0 1 1 0 0],[0 0 1 1 0])
  El Vigia II 230kV : PMComponent  Tag=PSATblock  Description=Connection  PhysicalDomain=psatdomain  LeftPortType=p1  RightPortType=p1  LConnTagsString=__newl0|__newl1  RConnTagsString=__newr0|__newr1  mask(Bus){in=2, out=2, p2q=230, p3_4q=[1.0419    -0.70804], p5q=1, p6q=1}
      mask prompts: in "Number of inputs:"; out "Number of outputs:"; p2q "Voltage Rating [kV]"; p3_4q "Voltage initial guess [p.u.  rad]"; p5q "Area number"; p6q "Region number"
      mask help: Bus block.
      mask init:
      | fm_inout
      settings: AttributesFormatString="|V| =  0.8952 p.u.\\n<V  =  0.2392 rad"
      mask CallbackString: ||||fm_block|
      mask Display: plot([0 1 1 0 0],[0 0 1 1 0])
  Furrial 230kV : PMComponent  Tag=PSATblock  Description=Connection  PhysicalDomain=psatdomain  LeftPortType=p1  RightPortType=p1  LConnTagsString=__newl0|__newl1  RConnTagsString=__newr0|__newr1|__newr2  mask(Bus){in=2, out=3, p2q=230, p3_4q=[1.0017     -0.2328], p5q=1, p6q=1}
      mask prompts: in "Number of inputs:"; out "Number of outputs:"; p2q "Voltage Rating [kV]"; p3_4q "Voltage initial guess [p.u.  rad]"; p5q "Area number"; p6q "Region number"
      mask help: Bus block.
      mask init:
      | fm_inout
      settings: AttributesFormatString="|V| =  0.9556 p.u.\\n<V  = -0.0986 rad"
      mask CallbackString: ||||fm_block|
      mask Display: plot([0 1 1 0 0],[0 0 1 1 0])
  Furrial 400kV : PMComponent  Tag=PSATblock  Description=Connection  PhysicalDomain=psatdomain  LeftPortType=p1  RightPortType=p1  LConnTagsString=__newl0|__newl1  RConnTagsString=__newr0|__newr1  mask(Bus){in=2, out=2, p2q=400, p3_4q=[0.99372    -0.23808], p5q=1, p6q=1}
      mask prompts: in "Number of inputs:"; out "Number of outputs:"; p2q "Voltage Rating [kV]"; p3_4q "Voltage initial guess [p.u.  rad]"; p5q "Area number"; p6q "Region number"
      mask help: Bus block.
      mask init:
      | fm_inout
      settings: AttributesFormatString="|V| =  0.9490 p.u.\\n<V  = -0.1799 rad"
      mask CallbackString: ||||fm_block|
      mask Display: plot([0 1 1 0 0],[0 0 1 1 0])
  Gen. Anz 2012-1 : PMComponent  Tag=PSATblock  Description=Connection  PhysicalDomain=psatdomain  LeftPortType=p1  RightPortType=p1  LConnTagsString=__newl0  RConnTagsString=__newr0  mask(Bus){in=1, out=1, p2q=400, p3_4q=[1 0], p5q=1, p6q=1}
      mask prompts: in "Number of inputs:"; out "Number of outputs:"; p2q "Voltage Rating [kV]"; p3_4q "Voltage initial guess [p.u.  rad]"; p5q "Area number"; p6q "Region number"
      mask help: Bus block.
      mask init:
      | fm_inout
      settings: AttributesFormatString="|V| =  1.02   p.u.\\n<V  = -0.0606 rad"
      mask CallbackString: ||||fm_block|
      mask Display: plot([0 1 1 0 0],[0 0 1 1 0])
  Gen. Anz 2012-2 : PMComponent  Tag=PSATblock  Description=Connection  PhysicalDomain=psatdomain  LeftPortType=p1  RightPortType=p1  LConnTagsString=__newl0  RConnTagsString=__newr0  mask(Bus){in=1, out=1, p2q=400, p3_4q=[1 0], p5q=1, p6q=1}
      mask prompts: in "Number of inputs:"; out "Number of outputs:"; p2q "Voltage Rating [kV]"; p3_4q "Voltage initial guess [p.u.  rad]"; p5q "Area number"; p6q "Region number"
      mask help: Bus block.
      mask init:
      | fm_inout
      settings: AttributesFormatString="|V| =  1.02   p.u.\\n<V  = -0.0311 rad"
      mask CallbackString: ||||fm_block|
      mask Display: plot([0 1 1 0 0],[0 0 1 1 0])
  Gen. Barinas 1 : PMComponent  Tag=PSATblock  Description=Connection  PhysicalDomain=psatdomain  LeftPortType=p1  RightPortType=p1  LConnTagsString=__newl0  RConnTagsString=__newr0  mask(Bus){in=1, out=1, p2q=230, p3_4q=[1 0], p5q=1, p6q=1}
      mask prompts: in "Number of inputs:"; out "Number of outputs:"; p2q "Voltage Rating [kV]"; p3_4q "Voltage initial guess [p.u.  rad]"; p5q "Area number"; p6q "Region number"
      mask help: Bus block.
      mask init:
      | fm_inout
      settings: AttributesFormatString="|V| =  1.02   p.u.\\n<V  = -0.2212 rad"
      mask CallbackString: ||||fm_block|
      mask Display: plot([0 1 1 0 0],[0 0 1 1 0])
  Gen. Barinas 2012 : PMComponent  Tag=PSATblock  Description=Connection  PhysicalDomain=psatdomain  LeftPortType=p1  RightPortType=p1  LConnTagsString=__newl0  RConnTagsString=__newr0  mask(Bus){in=1, out=1, p2q=230, p3_4q=[1 0], p5q=1, p6q=1}
      mask prompts: in "Number of inputs:"; out "Number of outputs:"; p2q "Voltage Rating [kV]"; p3_4q "Voltage initial guess [p.u.  rad]"; p5q "Area number"; p6q "Region number"
      mask help: Bus block.
      mask init:
      | fm_inout
      settings: AttributesFormatString="|V| =  1.02   p.u.\\n<V  = -0.2212 rad"
      mask CallbackString: ||||fm_block|
      mask Display: plot([0 1 1 0 0],[0 0 1 1 0])
  Gen. Guarico 2012 : PMComponent  Tag=PSATblock  Description=Connection  PhysicalDomain=psatdomain  LeftPortType=p1  RightPortType=p1  LConnTagsString=__newl0  RConnTagsString=__newr0  mask(Bus){in=1, out=1, p2q=230, p3_4q=[1.0021    -0.55915], p5q=1, p6q=1}
      mask prompts: in "Number of inputs:"; out "Number of outputs:"; p2q "Voltage Rating [kV]"; p3_4q "Voltage initial guess [p.u.  rad]"; p5q "Area number"; p6q "Region number"
      mask help: Bus block.
      mask init:
      | fm_inout
      settings: AttributesFormatString="|V| =  1.02   p.u.\\n<V  = -0.2650 rad"
      mask CallbackString: ||||fm_block|
      mask Display: plot([0 1 1 0 0],[0 0 1 1 0])
  Gen. Miranda 2012 : PMComponent  Tag=PSATblock  Description=Connection  PhysicalDomain=psatdomain  LeftPortType=p1  RightPortType=p1  LConnTagsString=__newl0  RConnTagsString=__newr0  mask(Bus){in=1, out=1, p2q=230, p3_4q=[1 0], p5q=1, p6q=1}
      mask prompts: in "Number of inputs:"; out "Number of outputs:"; p2q "Voltage Rating [kV]"; p3_4q "Voltage initial guess [p.u.  rad]"; p5q "Area number"; p6q "Region number"
      mask help: Bus block.
      mask init:
      | fm_inout
      settings: AttributesFormatString="|V| =  1.02   p.u.\\n<V  = -0.2212 rad"
      mask CallbackString: ||||fm_block|
      mask Display: plot([0 1 1 0 0],[0 0 1 1 0])
  Guanta II 115kV : PMComponent  Tag=PSATblock  Description=Connection  PhysicalDomain=psatdomain  LeftPortType=p1  RightPortType=p1  LConnTagsString=__newl0|__newl1  RConnTagsString=__newr0  mask(Bus){in=2, out=1, p2q=115, p3_4q=[1.0023    -0.25717], p5q=1, p6q=1}
      mask prompts: in "Number of inputs:"; out "Number of outputs:"; p2q "Voltage Rating [kV]"; p3_4q "Voltage initial guess [p.u.  rad]"; p5q "Area number"; p6q "Region number"
      mask help: Bus block.
      mask init:
      | fm_inout
      settings: AttributesFormatString="|V| =  0.9867 p.u.\\n<V  =  0.0450 rad"
      mask CallbackString: ||||fm_block|
      mask Display: plot([0 1 1 0 0],[0 0 1 1 0])
  Guanta II 230kV : PMComponent  Tag=PSATblock  Description=Connection  PhysicalDomain=psatdomain  LeftPortType=p1  RightPortType=p1  LConnTagsString=__newl0|__newl1|__newl2|__newl3  RConnTagsString=__newr0|__newr1|__newr2|__newr3  mask(Bus){in=4, out=4, p2q=230, p3_4q=[1.02    -0.24902], p5q=1, p6q=1}
      mask prompts: in "Number of inputs:"; out "Number of outputs:"; p2q "Voltage Rating [kV]"; p3_4q "Voltage initial guess [p.u.  rad]"; p5q "Area number"; p6q "Region number"
      mask help: Bus block.
      mask init:
      | fm_inout
      settings: AttributesFormatString="|V| =  1.02   p.u.\\n<V  =  0.0471 rad"
      mask CallbackString: ||||fm_block|
      mask Display: plot([0 1 1 0 0],[0 0 1 1 0])
  Guayana A : PMComponent  Tag=PSATblock  Description=Connection  PhysicalDomain=psatdomain  LeftPortType=p1  RightPortType=p1  LConnTagsString=__newl0|__newl1|__newl2|__newl3  RConnTagsString=__newr0|__newr1  mask(Bus){in=4, out=2, p2q=230, p3_4q=[1.07    -0.19263], p5q=1, p6q=1}
      mask prompts: in "Number of inputs:"; out "Number of outputs:"; p2q "Voltage Rating [kV]"; p3_4q "Voltage initial guess [p.u.  rad]"; p5q "Area number"; p6q "Region number"
      mask help: Bus block.
      mask init:
      | fm_inout
      settings: AttributesFormatString="|V| =  1.03   p.u.\\n<V  = -0.0247 rad"
      mask CallbackString: ||||fm_block|
      mask Display: plot([0 1 1 0 0],[0 0 1 1 0])
  Guayana B : PMComponent  Tag=PSATblock  Description=Connection  PhysicalDomain=psatdomain  LeftPortType=p1  RightPortType=p1  LConnTagsString=__newl0|__newl1|__newl2|__newl3  RConnTagsString=__newr0|__newr1  mask(Bus){in=4, out=2, p2q=400, p3_4q=[1.0142    -0.15088], p5q=1, p6q=1}
      mask prompts: in "Number of inputs:"; out "Number of outputs:"; p2q "Voltage Rating [kV]"; p3_4q "Voltage initial guess [p.u.  rad]"; p5q "Area number"; p6q "Region number"
      mask help: Bus block.
      mask init:
      | fm_inout
      settings: AttributesFormatString="|V| =  0.9722 p.u.\\n<V  = -0.1393 rad"
      mask CallbackString: ||||fm_block|
      mask Display: plot([0 1 1 0 0],[0 0 1 1 0])
  Guri 230kV : PMComponent  Tag=PSATblock  Description=Connection  PhysicalDomain=psatdomain  LeftPortType=p1  RightPortType=p1  LConnTagsString=__newl0|__newl1|__newl2  RConnTagsString=__newr0  mask(Bus){in=3, out=1, p2q=230, p3_4q=[1.0719    -0.13773], p5q=1, p6q=1}
      mask prompts: in "Number of inputs:"; out "Number of outputs:"; p2q "Voltage Rating [kV]"; p3_4q "Voltage initial guess [p.u.  rad]"; p5q "Area number"; p6q "Region number"
      mask help: Bus block.
      mask init:
      | fm_inout
      settings: AttributesFormatString="|V| =  1.05   p.u.\\n<V  =  0.0436 rad"
      mask CallbackString: ||||fm_block|
      mask Display: plot([0 1 1 0 0],[0 0 1 1 0])
  Guri 400kV A : PMComponent  Tag=PSATblock  Description=Connection  PhysicalDomain=psatdomain  LeftPortType=p1  RightPortType=p1  LConnTagsString=__newl0|__newl1|__newl2|__newl3|__newl4|__newl5  RConnTagsString=__newr0|__newr1  mask(Bus){in=6, out=2, p2q=400, p3_4q=[1.07    -0.05981], p5q=1, p6q=1}
      mask prompts: in "Number of inputs:"; out "Number of outputs:"; p2q "Voltage Rating [kV]"; p3_4q "Voltage initial guess [p.u.  rad]"; p5q "Area number"; p6q "Region number"
      mask help: Bus block.
      mask init:
      | fm_inout
      settings: AttributesFormatString="|V| =  1.05   p.u.\\n<V  =  0.0101 rad"
      mask CallbackString: ||||fm_block|
      mask Display: plot([0 1 1 0 0],[0 0 1 1 0])
  Guri 400kV B : PMComponent  Tag=PSATblock  Description=Connection  PhysicalDomain=psatdomain  LeftPortType=p1  RightPortType=p1  LConnTagsString=__newl0|__newl1|__newl2|__newl3  RConnTagsString=__newr0|__newr1|__newr2  mask(Bus){in=4, out=3, p2q=400, p3_4q=[1.0552   -0.050057], p5q=1, p6q=1}
      mask prompts: in "Number of inputs:"; out "Number of outputs:"; p2q "Voltage Rating [kV]"; p3_4q "Voltage initial guess [p.u.  rad]"; p5q "Area number"; p6q "Region number"
      mask help: Bus block.
      mask init:
      | fm_inout
      settings: AttributesFormatString="|V| =  1.0262 p.u.\\n<V  = -0.0362 rad"
      mask CallbackString: ||||fm_block|
      mask Display: plot([0 1 1 0 0],[0 0 1 1 0])
  Guri 765kV : PMComponent  Tag=PSATblock  Description=Connection  PhysicalDomain=psatdomain  LeftPortType=p1  RightPortType=p1  LConnTagsString=__newl0|__newl1|__newl2|__newl3|__newl4|__newl5  RConnTagsString=__newr0|__newr1|__newr2  mask(Bus){in=6, out=3, p2q=765, p3_4q=[1.07           0], p5q=1, p6q=1}
      mask prompts: in "Number of inputs:"; out "Number of outputs:"; p2q "Voltage Rating [kV]"; p3_4q "Voltage initial guess [p.u.  rad]"; p5q "Area number"; p6q "Region number"
      mask help: Bus block.
      mask init:
      | fm_inout
      settings: AttributesFormatString="|V| =  1.05   p.u.\\n<V  =  0      rad"
      mask CallbackString: ||||fm_block|
      mask Display: plot([0 1 1 0 0],[0 0 1 1 0])
  Isiro 115kV : PMComponent  Tag=PSATblock  Description=Connection  PhysicalDomain=psatdomain  LeftPortType=p1  RightPortType=p1  LConnTagsString=__newl0|__newl1|__newl2|__newl3  RConnTagsString=__newr0  mask(Bus){in=4, out=1, p2q=115, p3_4q=[0.95525    -0.20379], p5q=1, p6q=1}
      mask prompts: in "Number of inputs:"; out "Number of outputs:"; p2q "Voltage Rating [kV]"; p3_4q "Voltage initial guess [p.u.  rad]"; p5q "Area number"; p6q "Region number"
      mask help: Bus block.
      mask init:
      | fm_inout
      settings: AttributesFormatString="|V| =  0.9805 p.u.\\n<V  =  0.4136 rad"
      mask CallbackString: ||||fm_block|
      mask Display: plot([0 1 1 0 0],[0 0 1 1 0])
  Isiro 230kV : PMComponent  Tag=PSATblock  Description=Connection  PhysicalDomain=psatdomain  LeftPortType=p1  RightPortType=p1  LConnTagsString=__newl0|__newl1  RConnTagsString=__newr0|__newr1  mask(Bus){in=2, out=2, p2q=230, p3_4q=[0.97836    -0.32408], p5q=1, p6q=1}
      mask prompts: in "Number of inputs:"; out "Number of outputs:"; p2q "Voltage Rating [kV]"; p3_4q "Voltage initial guess [p.u.  rad]"; p5q "Area number"; p6q "Region number"
      mask help: Bus block.
      mask init:
      | fm_inout
      settings: AttributesFormatString="|V| =  0.9509 p.u.\\n<V  =  0.1465 rad"
      mask CallbackString: ||||fm_block|
      mask Display: plot([0 1 1 0 0],[0 0 1 1 0])
  Jose 400kV : PMComponent  Tag=PSATblock  Description=Connection  PhysicalDomain=psatdomain  LeftPortType=p1  RightPortType=p1  LConnTagsString=__newl0|__newl1  RConnTagsString=__newr0|__newr1|__newr2  mask(Bus){in=2, out=3, p2q=400, p3_4q=[1.0223    -0.26866], p5q=1, p6q=1}
      mask prompts: in "Number of inputs:"; out "Number of outputs:"; p2q "Voltage Rating [kV]"; p3_4q "Voltage initial guess [p.u.  rad]"; p5q "Area number"; p6q "Region number"
      mask help: Bus block.
      mask init:
      | fm_inout
      settings: AttributesFormatString="|V| =  1.0203 p.u.\\n<V  = -0.0651 rad"
      mask CallbackString: ||||fm_block|
      mask Display: plot([0 1 1 0 0],[0 0 1 1 0])
  Junquito 230kV : PMComponent  Tag=PSATblock  Description=Connection  PhysicalDomain=psatdomain  LeftPortType=p1  RightPortType=p1  LConnTagsString=__newl0|__newl1|__newl2  RConnTagsString=__newr0|__newr1  mask(Bus){in=3, out=2, p2q=230, p3_4q=[1.0104    -0.46538], p5q=1, p6q=1}
      mask prompts: in "Number of inputs:"; out "Number of outputs:"; p2q "Voltage Rating [kV]"; p3_4q "Voltage initial guess [p.u.  rad]"; p5q "Area number"; p6q "Region number"
      mask help: Bus block.
      mask init:
      | fm_inout
      settings: AttributesFormatString="|V| =  1.0225 p.u.\\n<V  = -0.2956 rad"
      mask CallbackString: ||||fm_block|
      mask Display: plot([0 1 1 0 0],[0 0 1 1 0])
  La Arenosa 230kV : PMComponent  Tag=PSATblock  Description=Connection  PhysicalDomain=psatdomain  LeftPortType=p1  RightPortType=p1  LConnTagsString=__newl0|__newl1|__newl2|__newl3|__newl4|__newl5|__newl6|__newl7  RConnTagsString=__newr0|__newr1|__newr2|__newr3|__newr4|__newr5|__newr6|__newr7  mask(Bus){in=8, out=8, p2q=230, p3_4q=[0.98578    -0.53261], p5q=1, p6q=1}
      mask prompts: in "Number of inputs:"; out "Number of outputs:"; p2q "Voltage Rating [kV]"; p3_4q "Voltage initial guess [p.u.  rad]"; p5q "Area number"; p6q "Region number"
      mask help: Bus block.
      mask init:
      | fm_inout
      settings: AttributesFormatString="|V| =  0.9937 p.u.\\n<V  = -0.3319 rad"
      mask CallbackString: ||||fm_block|
      mask Display: plot([0 1 1 0 0],[0 0 1 1 0])
  La Arenosa 400kV : PMComponent  Tag=PSATblock  Description=Connection  PhysicalDomain=psatdomain  LeftPortType=p1  RightPortType=p1  LConnTagsString=__newl0|__newl1|__newl2|__newl3|__newl4|__newl5  RConnTagsString=__newr0|__newr1  mask(Bus){in=6, out=2, p2q=400, p3_4q=[0.97877     -0.4492], p5q=1, p6q=1}
      mask prompts: in "Number of inputs:"; out "Number of outputs:"; p2q "Voltage Rating [kV]"; p3_4q "Voltage initial guess [p.u.  rad]"; p5q "Area number"; p6q "Region number"
      mask help: Bus block.
      mask init:
      | fm_inout
      settings: AttributesFormatString="|V| =  0.9783 p.u.\\n<V  = -0.2344 rad"
      mask CallbackString: ||||fm_block|
      mask Display: plot([0 1 1 0 0],[0 0 1 1 0])
  La Arenosa 765kV : PMComponent  Tag=PSATblock  Description=Connection  PhysicalDomain=psatdomain  LeftPortType=p1  RightPortType=p1  LConnTagsString=__newl0|__newl1  RConnTagsString=__newr0|__newr1|__newr2|__newr3|__newr4  mask(Bus){in=2, out=5, p2q=765, p3_4q=[0.99847    -0.42871], p5q=1, p6q=1}
      mask prompts: in "Number of inputs:"; out "Number of outputs:"; p2q "Voltage Rating [kV]"; p3_4q "Voltage initial guess [p.u.  rad]"; p5q "Area number"; p6q "Region number"
      mask help: Bus block.
      mask init:
      | fm_inout
      settings: AttributesFormatString="|V| =  1.0118 p.u.\\n<V  = -0.2528 rad"
      mask CallbackString: ||||fm_block|
      mask Display: plot([0 1 1 0 0],[0 0 1 1 0])
  La Canoa 400kV : PMComponent  Tag=PSATblock  Description=Connection  PhysicalDomain=psatdomain  LeftPortType=p1  RightPortType=p1  LConnTagsString=__newl0|__newl1  RConnTagsString=__newr0  mask(Bus){in=2, out=1, p2q=400, p3_4q=[1.0615    -0.13875], p5q=1, p6q=1}
      mask prompts: in "Number of inputs:"; out "Number of outputs:"; p2q "Voltage Rating [kV]"; p3_4q "Voltage initial guess [p.u.  rad]"; p5q "Area number"; p6q "Region number"
      mask help: Bus block.
      mask init:
      | fm_inout
      settings: AttributesFormatString="|V| =  1.0398 p.u.\\n<V  = -0.0227 rad"
      mask CallbackString: ||||fm_block|
      mask Display: plot([0 1 1 0 0],[0 0 1 1 0])
  La Horqueta 230kV : PMComponent  Tag=PSATblock  Description=Connection  PhysicalDomain=psatdomain  LeftPortType=p1  RightPortType=p1  LConnTagsString=__newl0|__newl1|__newl2|__newl3|__newl4|__newl5|__newl6|__newl7  RConnTagsString=__newr0|__newr1|__newr2|__newr3|__newr4  mask(Bus){in=8, out=5, p2q=230, p3_4q=[0.98199    -0.50182], p5q=1, p6q=1}
      mask prompts: in "Number of inputs:"; out "Number of outputs:"; p2q "Voltage Rating [kV]"; p3_4q "Voltage initial guess [p.u.  rad]"; p5q "Area number"; p6q "Region number"
      mask help: Bus block.
      mask init:
      | fm_inout
      settings: AttributesFormatString="|V| =  1.007  p.u.\\n<V  = -0.311  rad"
      mask CallbackString: ||||fm_block|
      mask Display: plot([0 1 1 0 0],[0 0 1 1 0])
  La Horqueta 400kV : PMComponent  Tag=PSATblock  Description=Connection  PhysicalDomain=psatdomain  LeftPortType=p1  RightPortType=p1  LConnTagsString=__newl0|__newl1|__newl2|__newl3  RConnTagsString=__newr0|__newr1  mask(Bus){in=4, out=2, p2q=400, p3_4q=[1.002    -0.44264], p5q=1, p6q=1}
      mask prompts: in "Number of inputs:"; out "Number of outputs:"; p2q "Voltage Rating [kV]"; p3_4q "Voltage initial guess [p.u.  rad]"; p5q "Area number"; p6q "Region number"
      mask help: Bus block.
      mask init:
      | fm_inout
      settings: AttributesFormatString="|V| =  1.006  p.u.\\n<V  = -0.2486 rad"
      mask CallbackString: ||||fm_block|
      mask Display: plot([0 1 1 0 0],[0 0 1 1 0])
  La Horqueta 765kV : PMComponent  Tag=PSATblock  Description=Connection  PhysicalDomain=psatdomain  LeftPortType=p1  RightPortType=p1  LConnTagsString=__newl0|__newl1  RConnTagsString=__newr0|__newr1|__newr2|__newr3  mask(Bus){in=2, out=4, p2q=765, p3_4q=[1.05    -0.39644], p5q=1, p6q=1}
      mask prompts: in "Number of inputs:"; out "Number of outputs:"; p2q "Voltage Rating [kV]"; p3_4q "Voltage initial guess [p.u.  rad]"; p5q "Area number"; p6q "Region number"
      mask help: Bus block.
      mask init:
      | fm_inout
      settings: AttributesFormatString="|V| =  1.05   p.u.\\n<V  = -0.2337 rad"
      mask CallbackString: ||||fm_block|
      mask Display: plot([0 1 1 0 0],[0 0 1 1 0])
  Las Claritas 230kV : PMComponent  Tag=PSATblock  Description=Connection  PhysicalDomain=psatdomain  LeftPortType=p1  RightPortType=p1  LConnTagsString=__newl0  RConnTagsString=__newr0  mask(Bus){in=1, out=1, p2q=230, p3_4q=[1.0094    -0.18727], p5q=1, p6q=1}
      mask prompts: in "Number of inputs:"; out "Number of outputs:"; p2q "Voltage Rating [kV]"; p3_4q "Voltage initial guess [p.u.  rad]"; p5q "Area number"; p6q "Region number"
      mask help: Bus block.
      mask init:
      | fm_inout
      settings: AttributesFormatString="|V| =  1.0018 p.u.\\n<V  = -0.1835 rad"
      mask CallbackString: ||||fm_block|
      mask Display: plot([0 1 1 0 0],[0 0 1 1 0])
  Las Claritas 400kV : PMComponent  Tag=PSATblock  Description=Connection  PhysicalDomain=psatdomain  LeftPortType=p1  RightPortType=p1  LConnTagsString=__newl0|__newl1  RConnTagsString=__newr0  mask(Bus){in=2, out=1, p2q=400, p3_4q=[1.146    -0.14257], p5q=1, p6q=1}
      mask prompts: in "Number of inputs:"; out "Number of outputs:"; p2q "Voltage Rating [kV]"; p3_4q "Voltage initial guess [p.u.  rad]"; p5q "Area number"; p6q "Region number"
      mask help: Bus block.
      mask init:
      | fm_inout
      settings: AttributesFormatString="|V| =  1.0947 p.u.\\n<V  = -0.1353 rad"
      mask CallbackString: ||||fm_block|
      mask Display: plot([0 1 1 0 0],[0 0 1 1 0])
  Las Flores 230kV : PMComponent  Tag=PSATblock  Description=Connection  PhysicalDomain=psatdomain  LeftPortType=p1  RightPortType=p1  LConnTagsString=__newl0|__newl1  RConnTagsString=__newr0  mask(Bus){in=2, out=1, p2q=230, p3_4q=[1.0163    -0.62695], p5q=1, p6q=1}
      mask prompts: in "Number of inputs:"; out "Number of outputs:"; p2q "Voltage Rating [kV]"; p3_4q "Voltage initial guess [p.u.  rad]"; p5q "Area number"; p6q "Region number"
      mask help: Bus block.
      mask init:
      | fm_inout
      settings: AttributesFormatString="|V| =  1.0162 p.u.\\n<V  = -0.2778 rad"
      mask CallbackString: ||||fm_block|
      mask Display: plot([0 1 1 0 0],[0 0 1 1 0])
  Line : PMComponent  Tag=PSATblock  Description=Power Flow  PhysicalDomain=psatdomain  LeftPortType=p1  RightPortType=p1  LConnTagsString=__newl0  RConnTagsString=__newr0  mask(Line){p3_4_5q=[100 765 60], p6q=[161], p8q=[0.012], p9q=[0.0008727], p10q=[0.013204566e-6], p13_14_15q=[25.29 22.76 25.29], p16q=on}
      mask prompts: p3_4_5q "Power, Voltage and Frequency Ratings [MVA, kV, Hz]"; p6q "Length of line [km] (0 for p.u. parameters)"; p8q "Resistance [p.u. (Ohms/km)]"; p9q "Reactance [p.u. (H/km)]"; p10q "Susceptance [p.u. (F/km)]"; p13_14_15q "Imax, Pmax and Smax [p.u., p.u., p.u.]"; p16q "Connected"
      mask help: This block defines a pi model for a tree phase line.
      mask init:
      | [xp,yp] = fm_draw('pi');
      mask CallbackString: ||||||fm_block
      mask Display:
      | plot([-1  1  1 -1 -1],[-0.2 -0.2 0.2 0.2 -0.2])
      | color('blue')
      | plot(0.35*xp,0.2*yp)
  Line1 : PMComponent  Tag=PSATblock  Description=Power Flow  PhysicalDomain=psatdomain  LeftPortType=p1  RightPortType=p1  LConnTagsString=__newl0  RConnTagsString=__newr0  mask(Line){p3_4_5q=[100 765 60], p6q=[161], p8q=[0.012], p9q=[0.0008727], p10q=[0.013204566e-6], p13_14_15q=[25.29 22.76 25.29], p16q=on}
      mask prompts: p3_4_5q "Power, Voltage and Frequency Ratings [MVA, kV, Hz]"; p6q "Length of line [km] (0 for p.u. parameters)"; p8q "Resistance [p.u. (Ohms/km)]"; p9q "Reactance [p.u. (H/km)]"; p10q "Susceptance [p.u. (F/km)]"; p13_14_15q "Imax, Pmax and Smax [p.u., p.u., p.u.]"; p16q "Connected"
      mask help: This block defines a pi model for a tree phase line.
      mask init:
      | [xp,yp] = fm_draw('pi');
      mask CallbackString: ||||||fm_block
      mask Display:
      | plot([-1  1  1 -1 -1],[-0.2 -0.2 0.2 0.2 -0.2])
      | color('blue')
      | plot(0.35*xp,0.2*yp)
  Line10 : PMComponent  Tag=PSATblock  Description=Power Flow  PhysicalDomain=psatdomain  LeftPortType=p1  RightPortType=p1  LConnTagsString=__newl0  RConnTagsString=__newr0  mask(Line){p3_4_5q=[100  230  60], p6q=43.6, p8q=[0.05], p9q=[0.001294461], p10q=[0.008941863e-6], p13_14_15q=[27.3 24.9 27.3], p16q=on}
      mask prompts: p3_4_5q "Power, Voltage and Frequency Ratings [MVA, kV, Hz]"; p6q "Length of line [km] (0 for p.u. parameters)"; p8q "Resistance [p.u. (Ohms/km)]"; p9q "Reactance [p.u. (H/km)]"; p10q "Susceptance [p.u. (F/km)]"; p13_14_15q "Imax, Pmax and Smax [p.u., p.u., p.u.]"; p16q "Connected"
      mask help: This block defines a pi model for a tree phase line.
      mask init:
      | [xp,yp] = fm_draw('pi');
      mask CallbackString: ||||||fm_block
      mask Display:
      | plot([-1  1  1 -1 -1],[-0.2 -0.2 0.2 0.2 -0.2])
      | color('blue')
      | plot(0.35*xp,0.2*yp)
  Line100 : PMComponent  Tag=PSATblock  Description=Power Flow  PhysicalDomain=psatdomain  LeftPortType=p1  RightPortType=p1  LConnTagsString=__newl0  RConnTagsString=__newr0  mask(Line){p3_4_5q=[100  230  60], p6q=109, p8q=[0.05], p9q=[0.001294461], p10q=[0.008941863e-6], p13_14_15q=[10.9 9.9 10.9], p16q=on}
      mask prompts: p3_4_5q "Power, Voltage and Frequency Ratings [MVA, kV, Hz]"; p6q "Length of line [km] (0 for p.u. parameters)"; p8q "Resistance [p.u. (Ohms/km)]"; p9q "Reactance [p.u. (H/km)]"; p10q "Susceptance [p.u. (F/km)]"; p13_14_15q "Imax, Pmax and Smax [p.u., p.u., p.u.]"; p16q "Connected"
      mask help: This block defines a pi model for a tree phase line.
      mask init:
      | [xp,yp] = fm_draw('pi');
      mask CallbackString: ||||||fm_block
      mask Display:
      | plot([-1  1  1 -1 -1],[-0.2 -0.2 0.2 0.2 -0.2])
      | color('blue')
      | plot(0.35*xp,0.2*yp)
  Line101 : PMComponent  Tag=PSATblock  Description=Power Flow  PhysicalDomain=psatdomain  LeftPortType=p1  RightPortType=p1  LConnTagsString=__newl0  RConnTagsString=__newr0  mask(Line){p3_4_5q=[100  400  60], p6q=187, p8q=[0.033806452], p9q=[0.000933966], p10q=[0.012626303e-6], p13_14_15q=[26.7 24.3 26.7], p16q=on}
      mask prompts: p3_4_5q "Power, Voltage and Frequency Ratings [MVA, kV, Hz]"; p6q "Length of line [km] (0 for p.u. parameters)"; p8q "Resistance [p.u. (Ohms/km)]"; p9q "Reactance [p.u. (H/km)]"; p10q "Susceptance [p.u. (F/km)]"; p13_14_15q "Imax, Pmax and Smax [p.u., p.u., p.u.]"; p16q "Connected"
      mask help: This block defines a pi model for a tree phase line.
      mask init:
      | [xp,yp] = fm_draw('pi');
      mask CallbackString: ||||||fm_block
      mask Display:
      | plot([-1  1  1 -1 -1],[-0.2 -0.2 0.2 0.2 -0.2])
      | color('blue')
      | plot(0.35*xp,0.2*yp)
  Line102 : PMComponent  Tag=PSATblock  Description=Power Flow  PhysicalDomain=psatdomain  LeftPortType=p1  RightPortType=p1  LConnTagsString=__newl0  RConnTagsString=__newr0  mask(Line){p3_4_5q=[100  230  60], p6q=130, p8q=[0.05], p9q=[0.001294461], p10q=[0.008941863e-6], p13_14_15q=[9.2 8.3 9.2], p16q=on}
      mask prompts: p3_4_5q "Power, Voltage and Frequency Ratings [MVA, kV, Hz]"; p6q "Length of line [km] (0 for p.u. parameters)"; p8q "Resistance [p.u. (Ohms/km)]"; p9q "Reactance [p.u. (H/km)]"; p10q "Susceptance [p.u. (F/km)]"; p13_14_15q "Imax, Pmax and Smax [p.u., p.u., p.u.]"; p16q "Connected"
      mask help: This block defines a pi model for a tree phase line.
      mask init:
      | [xp,yp] = fm_draw('pi');
      mask CallbackString: ||||||fm_block
      mask Display:
      | plot([-1  1  1 -1 -1],[-0.2 -0.2 0.2 0.2 -0.2])
      | color('blue')
      | plot(0.35*xp,0.2*yp)
  Line103 : PMComponent  Tag=PSATblock  Description=Power Flow  PhysicalDomain=psatdomain  LeftPortType=p1  RightPortType=p1  LConnTagsString=__newl0  RConnTagsString=__newr0  mask(Line){p3_4_5q=[100  230  60], p6q=300, p8q=[0.05], p9q=[0.001294461], p10q=[0.008941863e-6], p13_14_15q=[4 3.6 4], p16q=on}
      mask prompts: p3_4_5q "Power, Voltage and Frequency Ratings [MVA, kV, Hz]"; p6q "Length of line [km] (0 for p.u. parameters)"; p8q "Resistance [p.u. (Ohms/km)]"; p9q "Reactance [p.u. (H/km)]"; p10q "Susceptance [p.u. (F/km)]"; p13_14_15q "Imax, Pmax and Smax [p.u., p.u., p.u.]"; p16q "Connected"
      mask help: This block defines a pi model for a tree phase line.
      mask init:
      | [xp,yp] = fm_draw('pi');
      mask CallbackString: ||||||fm_block
      mask Display:
      | plot([-1  1  1 -1 -1],[-0.2 -0.2 0.2 0.2 -0.2])
      | color('blue')
      | plot(0.35*xp,0.2*yp)
  Line104 : PMComponent  Tag=PSATblock  Description=Power Flow  PhysicalDomain=psatdomain  LeftPortType=p1  RightPortType=p1  LConnTagsString=__newl0  RConnTagsString=__newr0  mask(Line){p3_4_5q=[100  230  60], p6q=300, p8q=[0.05], p9q=[0.001294461], p10q=[0.008941863e-6], p13_14_15q=[4 3.6 4], p16q=on}
      mask prompts: p3_4_5q "Power, Voltage and Frequency Ratings [MVA, kV, Hz]"; p6q "Length of line [km] (0 for p.u. parameters)"; p8q "Resistance [p.u. (Ohms/km)]"; p9q "Reactance [p.u. (H/km)]"; p10q "Susceptance [p.u. (F/km)]"; p13_14_15q "Imax, Pmax and Smax [p.u., p.u., p.u.]"; p16q "Connected"
      mask help: This block defines a pi model for a tree phase line.
      mask init:
      | [xp,yp] = fm_draw('pi');
      mask CallbackString: ||||||fm_block
      mask Display:
      | plot([-1  1  1 -1 -1],[-0.2 -0.2 0.2 0.2 -0.2])
      | color('blue')
      | plot(0.35*xp,0.2*yp)
  Line105 : PMComponent  Tag=PSATblock  Description=Power Flow  PhysicalDomain=psatdomain  LeftPortType=p1  RightPortType=p1  LConnTagsString=__newl0  RConnTagsString=__newr0  mask(Line){p3_4_5q=[100  230  60], p6q=68, p8q=[0.05], p9q=[0.001294461], p10q=[0.008941863e-6], p13_14_15q=[17.5 15.9 17.5], p16q=on}
      mask prompts: p3_4_5q "Power, Voltage and Frequency Ratings [MVA, kV, Hz]"; p6q "Length of line [km] (0 for p.u. parameters)"; p8q "Resistance [p.u. (Ohms/km)]"; p9q "Reactance [p.u. (H/km)]"; p10q "Susceptance [p.u. (F/km)]"; p13_14_15q "Imax, Pmax and Smax [p.u., p.u., p.u.]"; p16q "Connected"
      mask help: This block defines a pi model for a tree phase line.
      mask init:
      | [xp,yp] = fm_draw('pi');
      mask CallbackString: ||||||fm_block
      mask Display:
      | plot([-1  1  1 -1 -1],[-0.2 -0.2 0.2 0.2 -0.2])
      | color('blue')
      | plot(0.35*xp,0.2*yp)
  Line106 : PMComponent  Tag=PSATblock  Description=Power Flow  PhysicalDomain=psatdomain  LeftPortType=p1  RightPortType=p1  LConnTagsString=__newl0  RConnTagsString=__newr0  mask(Line){p3_4_5q=[100  230  60], p6q=25, p8q=[0.05], p9q=[0.001294461], p10q=[0.008941863e-6], p13_14_15q=[47.7 43.4 47.7], p16q=on}
      mask prompts: p3_4_5q "Power, Voltage and Frequency Ratings [MVA, kV, Hz]"; p6q "Length of line [km] (0 for p.u. parameters)"; p8q "Resistance [p.u. (Ohms/km)]"; p9q "Reactance [p.u. (H/km)]"; p10q "Susceptance [p.u. (F/km)]"; p13_14_15q "Imax, Pmax and Smax [p.u., p.u., p.u.]"; p16q "Connected"
      mask help: This block defines a pi model for a tree phase line.
      mask init:
      | [xp,yp] = fm_draw('pi');
      mask CallbackString: ||||||fm_block
      mask Display:
      | plot([-1  1  1 -1 -1],[-0.2 -0.2 0.2 0.2 -0.2])
      | color('blue')
      | plot(0.35*xp,0.2*yp)
  Line107 : PMComponent  Tag=PSATblock  Description=Power Flow  PhysicalDomain=psatdomain  LeftPortType=p1  RightPortType=p1  LConnTagsString=__newl0  RConnTagsString=__newr0  mask(Line){p3_4_5q=[100  230  60], p6q=152, p8q=[0.05], p9q=|, p10q=[0.008941863e-6], p13_14_15q=[7.8 7.1 7.8], p16q=on}
      mask p9q=|
      | [0.001294461
      | ]
      mask prompts: p3_4_5q "Power, Voltage and Frequency Ratings [MVA, kV, Hz]"; p6q "Length of line [km] (0 for p.u. parameters)"; p8q "Resistance [p.u. (Ohms/km)]"; p9q "Reactance [p.u. (H/km)]"; p10q "Susceptance [p.u. (F/km)]"; p13_14_15q "Imax, Pmax and Smax [p.u., p.u., p.u.]"; p16q "Connected"
      mask help: This block defines a pi model for a tree phase line.
      mask init:
      | [xp,yp] = fm_draw('pi');
      mask CallbackString: ||||||fm_block
      mask Display:
      | plot([-1  1  1 -1 -1],[-0.2 -0.2 0.2 0.2 -0.2])
      | color('blue')
      | plot(0.35*xp,0.2*yp)
  Line108 : PMComponent  Tag=PSATblock  Description=Power Flow  PhysicalDomain=psatdomain  LeftPortType=p1  RightPortType=p1  LConnTagsString=__newl0  RConnTagsString=__newr0  mask(Line){p3_4_5q=[100  230  60], p6q=152, p8q=[0.05], p9q=|, p10q=[0.008941863e-6], p13_14_15q=[7.8 7.1 7.8], p16q=on}
      mask p9q=|
      | [0.001294461
      | ]
      mask prompts: p3_4_5q "Power, Voltage and Frequency Ratings [MVA, kV, Hz]"; p6q "Length of line [km] (0 for p.u. parameters)"; p8q "Resistance [p.u. (Ohms/km)]"; p9q "Reactance [p.u. (H/km)]"; p10q "Susceptance [p.u. (F/km)]"; p13_14_15q "Imax, Pmax and Smax [p.u., p.u., p.u.]"; p16q "Connected"
      mask help: This block defines a pi model for a tree phase line.
      mask init:
      | [xp,yp] = fm_draw('pi');
      mask CallbackString: ||||||fm_block
      mask Display:
      | plot([-1  1  1 -1 -1],[-0.2 -0.2 0.2 0.2 -0.2])
      | color('blue')
      | plot(0.35*xp,0.2*yp)
  Line109 : PMComponent  Tag=PSATblock  Description=Power Flow  PhysicalDomain=psatdomain  LeftPortType=p1  RightPortType=p1  LConnTagsString=__newl0  RConnTagsString=__newr0  mask(Line){p3_4_5q=[100  230  60], p6q=150, p8q=[0.05], p9q=[0.001294461], p10q=[0.008941863e-6], p13_14_15q=[7.9 7.2 7.9], p16q=on}
      mask prompts: p3_4_5q "Power, Voltage and Frequency Ratings [MVA, kV, Hz]"; p6q "Length of line [km] (0 for p.u. parameters)"; p8q "Resistance [p.u. (Ohms/km)]"; p9q "Reactance [p.u. (H/km)]"; p10q "Susceptance [p.u. (F/km)]"; p13_14_15q "Imax, Pmax and Smax [p.u., p.u., p.u.]"; p16q "Connected"
      mask help: This block defines a pi model for a tree phase line.
      mask init:
      | [xp,yp] = fm_draw('pi');
      mask CallbackString: ||||||fm_block
      mask Display:
      | plot([-1  1  1 -1 -1],[-0.2 -0.2 0.2 0.2 -0.2])
      | color('blue')
      | plot(0.35*xp,0.2*yp)
  Line11 : PMComponent  Tag=PSATblock  Description=Power Flow  PhysicalDomain=psatdomain  LeftPortType=p1  RightPortType=p1  LConnTagsString=__newl0  RConnTagsString=__newr0  mask(Line){p3_4_5q=[100  400  60], p6q=144.2, p8q=[0.033806452], p9q=[0.000933966], p10q=[0.012626303e-6], p13_14_15q=[34.7 31.5 34.7], p16q=on}
      mask prompts: p3_4_5q "Power, Voltage and Frequency Ratings [MVA, kV, Hz]"; p6q "Length of line [km] (0 for p.u. parameters)"; p8q "Resistance [p.u. (Ohms/km)]"; p9q "Reactance [p.u. (H/km)]"; p10q "Susceptance [p.u. (F/km)]"; p13_14_15q "Imax, Pmax and Smax [p.u., p.u., p.u.]"; p16q "Connected"
      mask help: This block defines a pi model for a tree phase line.
      mask init:
      | [xp,yp] = fm_draw('pi');
      mask CallbackString: ||||||fm_block
      mask Display:
      | plot([-1  1  1 -1 -1],[-0.2 -0.2 0.2 0.2 -0.2])
      | color('blue')
      | plot(0.35*xp,0.2*yp)
  Line110 : PMComponent  Tag=PSATblock  Description=Power Flow  PhysicalDomain=psatdomain  LeftPortType=p1  RightPortType=p1  LConnTagsString=__newl0  RConnTagsString=__newr0  mask(Line){p3_4_5q=[100  230  60], p6q=134, p8q=[0.05], p9q=[0.001294461], p10q=[0.008941863e-6], p13_14_15q=[8.9 8.1 8.9], p16q=on}
      mask prompts: p3_4_5q "Power, Voltage and Frequency Ratings [MVA, kV, Hz]"; p6q "Length of line [km] (0 for p.u. parameters)"; p8q "Resistance [p.u. (Ohms/km)]"; p9q "Reactance [p.u. (H/km)]"; p10q "Susceptance [p.u. (F/km)]"; p13_14_15q "Imax, Pmax and Smax [p.u., p.u., p.u.]"; p16q "Connected"
      mask help: This block defines a pi model for a tree phase line.
      mask init:
      | [xp,yp] = fm_draw('pi');
      mask CallbackString: ||||||fm_block
      mask Display:
      | plot([-1  1  1 -1 -1],[-0.2 -0.2 0.2 0.2 -0.2])
      | color('blue')
      | plot(0.35*xp,0.2*yp)
  Line111 : PMComponent  Tag=PSATblock  Description=Power Flow  PhysicalDomain=psatdomain  LeftPortType=p1  RightPortType=p1  LConnTagsString=__newl0  RConnTagsString=__newr0  mask(Line){p3_4_5q=[100  230  60], p6q=80, p8q=[0.05], p9q=[0.001294461], p10q=[0.008941863e-6], p13_14_15q=[14.9 13.6 14.9], p16q=on}
      mask prompts: p3_4_5q "Power, Voltage and Frequency Ratings [MVA, kV, Hz]"; p6q "Length of line [km] (0 for p.u. parameters)"; p8q "Resistance [p.u. (Ohms/km)]"; p9q "Reactance [p.u. (H/km)]"; p10q "Susceptance [p.u. (F/km)]"; p13_14_15q "Imax, Pmax and Smax [p.u., p.u., p.u.]"; p16q "Connected"
      mask help: This block defines a pi model for a tree phase line.
      mask init:
      | [xp,yp] = fm_draw('pi');
      mask CallbackString: ||||||fm_block
      mask Display:
      | plot([-1  1  1 -1 -1],[-0.2 -0.2 0.2 0.2 -0.2])
      | color('blue')
      | plot(0.35*xp,0.2*yp)
  Line112 : PMComponent  Tag=PSATblock  Description=Power Flow  PhysicalDomain=psatdomain  LeftPortType=p1  RightPortType=p1  LConnTagsString=__newl0  RConnTagsString=__newr0  mask(Line){p3_4_5q=[100  230  60], p6q=50, p8q=[0.05], p9q=[0.001294461], p10q=[0.008941863e-6], p13_14_15q=[23.8 21.7 23.8], p16q=on}
      mask prompts: p3_4_5q "Power, Voltage and Frequency Ratings [MVA, kV, Hz]"; p6q "Length of line [km] (0 for p.u. parameters)"; p8q "Resistance [p.u. (Ohms/km)]"; p9q "Reactance [p.u. (H/km)]"; p10q "Susceptance [p.u. (F/km)]"; p13_14_15q "Imax, Pmax and Smax [p.u., p.u., p.u.]"; p16q "Connected"
      mask help: This block defines a pi model for a tree phase line.
      mask init:
      | [xp,yp] = fm_draw('pi');
      mask CallbackString: ||||||fm_block
      mask Display:
      | plot([-1  1  1 -1 -1],[-0.2 -0.2 0.2 0.2 -0.2])
      | color('blue')
      | plot(0.35*xp,0.2*yp)
  Line113 : PMComponent  Tag=PSATblock  Description=Power Flow  PhysicalDomain=psatdomain  LeftPortType=p1  RightPortType=p1  LConnTagsString=__newl0  RConnTagsString=__newr0  mask(Line){p3_4_5q=[100  230  60], p6q=67, p8q=[0.05], p9q=[0.001294461], p10q=[0.008941863e-6], p13_14_15q=[17.8 16.2 17.8], p16q=on}
      mask prompts: p3_4_5q "Power, Voltage and Frequency Ratings [MVA, kV, Hz]"; p6q "Length of line [km] (0 for p.u. parameters)"; p8q "Resistance [p.u. (Ohms/km)]"; p9q "Reactance [p.u. (H/km)]"; p10q "Susceptance [p.u. (F/km)]"; p13_14_15q "Imax, Pmax and Smax [p.u., p.u., p.u.]"; p16q "Connected"
      mask help: This block defines a pi model for a tree phase line.
      mask init:
      | [xp,yp] = fm_draw('pi');
      mask CallbackString: ||||||fm_block
      mask Display:
      | plot([-1  1  1 -1 -1],[-0.2 -0.2 0.2 0.2 -0.2])
      | color('blue')
      | plot(0.35*xp,0.2*yp)
  Line114 : PMComponent  Tag=PSATblock  Description=Power Flow  PhysicalDomain=psatdomain  LeftPortType=p1  RightPortType=p1  LConnTagsString=__newl0  RConnTagsString=__newr0  mask(Line){p3_4_5q=[100  230  60], p6q=44, p8q=[0.05], p9q=[0.001294461], p10q=[0.008941863e-6], p13_14_15q=[27.1 24.6 27.1], p16q=on}
      mask prompts: p3_4_5q "Power, Voltage and Frequency Ratings [MVA, kV, Hz]"; p6q "Length of line [km] (0 for p.u. parameters)"; p8q "Resistance [p.u. (Ohms/km)]"; p9q "Reactance [p.u. (H/km)]"; p10q "Susceptance [p.u. (F/km)]"; p13_14_15q "Imax, Pmax and Smax [p.u., p.u., p.u.]"; p16q "Connected"
      mask help: This block defines a pi model for a tree phase line.
      mask init:
      | [xp,yp] = fm_draw('pi');
      mask CallbackString: ||||||fm_block
      mask Display:
      | plot([-1  1  1 -1 -1],[-0.2 -0.2 0.2 0.2 -0.2])
      | color('blue')
      | plot(0.35*xp,0.2*yp)
  Line115 : PMComponent  Tag=PSATblock  Description=Power Flow  PhysicalDomain=psatdomain  LeftPortType=p1  RightPortType=p1  LConnTagsString=__newl0  RConnTagsString=__newr0  mask(Line){p3_4_5q=[100  230  60], p6q=80, p8q=[0.05], p9q=[0.001294461], p10q=[0.008941863e-6], p13_14_15q=[14.9 13.6 14.9], p16q=on}
      mask prompts: p3_4_5q "Power, Voltage and Frequency Ratings [MVA, kV, Hz]"; p6q "Length of line [km] (0 for p.u. parameters)"; p8q "Resistance [p.u. (Ohms/km)]"; p9q "Reactance [p.u. (H/km)]"; p10q "Susceptance [p.u. (F/km)]"; p13_14_15q "Imax, Pmax and Smax [p.u., p.u., p.u.]"; p16q "Connected"
      mask help: This block defines a pi model for a tree phase line.
      mask init:
      | [xp,yp] = fm_draw('pi');
      mask CallbackString: ||||||fm_block
      mask Display:
      | plot([-1  1  1 -1 -1],[-0.2 -0.2 0.2 0.2 -0.2])
      | color('blue')
      | plot(0.35*xp,0.2*yp)
  Line116 : PMComponent  Tag=PSATblock  Description=Power Flow  PhysicalDomain=psatdomain  LeftPortType=p1  RightPortType=p1  LConnTagsString=__newl0  RConnTagsString=__newr0  mask(Line){p3_4_5q=[100  230  60], p6q=13, p8q=[0.05], p9q=[0.001294461], p10q=[0.008941863e-6], p13_14_15q=[91.7 83.4 91.7], p16q=on}
      mask prompts: p3_4_5q "Power, Voltage and Frequency Ratings [MVA, kV, Hz]"; p6q "Length of line [km] (0 for p.u. parameters)"; p8q "Resistance [p.u. (Ohms/km)]"; p9q "Reactance [p.u. (H/km)]"; p10q "Susceptance [p.u. (F/km)]"; p13_14_15q "Imax, Pmax and Smax [p.u., p.u., p.u.]"; p16q "Connected"
      mask help: This block defines a pi model for a tree phase line.
      mask init:
      | [xp,yp] = fm_draw('pi');
      mask CallbackString: ||||||fm_block
      mask Display:
      | plot([-1  1  1 -1 -1],[-0.2 -0.2 0.2 0.2 -0.2])
      | color('blue')
      | plot(0.35*xp,0.2*yp)
  Line117 : PMComponent  Tag=PSATblock  Description=Power Flow  PhysicalDomain=psatdomain  LeftPortType=p1  RightPortType=p1  LConnTagsString=__newl0  RConnTagsString=__newr0  mask(Line){p3_4_5q=[100  230  60], p6q=133, p8q=[0.05], p9q=[0.001294461], p10q=[0.008941863e-6], p13_14_15q=[9 8.2 9], p16q=on}
      mask prompts: p3_4_5q "Power, Voltage and Frequency Ratings [MVA, kV, Hz]"; p6q "Length of line [km] (0 for p.u. parameters)"; p8q "Resistance [p.u. (Ohms/km)]"; p9q "Reactance [p.u. (H/km)]"; p10q "Susceptance [p.u. (F/km)]"; p13_14_15q "Imax, Pmax and Smax [p.u., p.u., p.u.]"; p16q "Connected"
      mask help: This block defines a pi model for a tree phase line.
      mask init:
      | [xp,yp] = fm_draw('pi');
      mask CallbackString: ||||||fm_block
      mask Display:
      | plot([-1  1  1 -1 -1],[-0.2 -0.2 0.2 0.2 -0.2])
      | color('blue')
      | plot(0.35*xp,0.2*yp)
  Line118 : PMComponent  Tag=PSATblock  Description=Power Flow  PhysicalDomain=psatdomain  LeftPortType=p1  RightPortType=p1  LConnTagsString=__newl0  RConnTagsString=__newr0  mask(Line){p3_4_5q=[100  230  60], p6q=95.4, p8q=[0.05], p9q=[0.001294461], p10q=[0.008941863e-6], p13_14_15q=[12.5 11.4 12.5], p16q=on}
      mask prompts: p3_4_5q "Power, Voltage and Frequency Ratings [MVA, kV, Hz]"; p6q "Length of line [km] (0 for p.u. parameters)"; p8q "Resistance [p.u. (Ohms/km)]"; p9q "Reactance [p.u. (H/km)]"; p10q "Susceptance [p.u. (F/km)]"; p13_14_15q "Imax, Pmax and Smax [p.u., p.u., p.u.]"; p16q "Connected"
      mask help: This block defines a pi model for a tree phase line.
      mask init:
      | [xp,yp] = fm_draw('pi');
      mask CallbackString: ||||||fm_block
      mask Display:
      | plot([-1  1  1 -1 -1],[-0.2 -0.2 0.2 0.2 -0.2])
      | color('blue')
      | plot(0.35*xp,0.2*yp)
  Line119 : PMComponent  Tag=PSATblock  Description=Power Flow  PhysicalDomain=psatdomain  LeftPortType=p1  RightPortType=p1  LConnTagsString=__newl0  RConnTagsString=__newr0  mask(Line){p3_4_5q=[532  230  60], p6q=224, p8q=[0.05], p9q=[0.001294461], p10q=[0.008941863e-6], p13_14_15q=[5.3 4.8 5.3], p16q=on}
      mask prompts: p3_4_5q "Power, Voltage and Frequency Ratings [MVA, kV, Hz]"; p6q "Length of line [km] (0 for p.u. parameters)"; p8q "Resistance [p.u. (Ohms/km)]"; p9q "Reactance [p.u. (H/km)]"; p10q "Susceptance [p.u. (F/km)]"; p13_14_15q "Imax, Pmax and Smax [p.u., p.u., p.u.]"; p16q "Connected"
      mask help: This block defines a pi model for a tree phase line.
      mask init:
      | [xp,yp] = fm_draw('pi');
      mask CallbackString: ||||||fm_block
      mask Display:
      | plot([-1  1  1 -1 -1],[-0.2 -0.2 0.2 0.2 -0.2])
      | color('blue')
      | plot(0.35*xp,0.2*yp)
  Line12 : PMComponent  Tag=PSATblock  Description=Power Flow  PhysicalDomain=psatdomain  LeftPortType=p1  RightPortType=p1  LConnTagsString=__newl0  RConnTagsString=__newr0  mask(Line){p3_4_5q=[100  400  60], p6q=153.9, p8q=[0.033806452], p9q=[0.000933966], p10q=[0.012626303e-6], p13_14_15q=[32.5 29.5 32.5], p16q=on}
      mask prompts: p3_4_5q "Power, Voltage and Frequency Ratings [MVA, kV, Hz]"; p6q "Length of line [km] (0 for p.u. parameters)"; p8q "Resistance [p.u. (Ohms/km)]"; p9q "Reactance [p.u. (H/km)]"; p10q "Susceptance [p.u. (F/km)]"; p13_14_15q "Imax, Pmax and Smax [p.u., p.u., p.u.]"; p16q "Connected"
      mask help: This block defines a pi model for a tree phase line.
      mask init:
      | [xp,yp] = fm_draw('pi');
      mask CallbackString: ||||||fm_block
      mask Display:
      | plot([-1  1  1 -1 -1],[-0.2 -0.2 0.2 0.2 -0.2])
      | color('blue')
      | plot(0.35*xp,0.2*yp)
  Line120 : PMComponent  Tag=PSATblock  Description=Power Flow  PhysicalDomain=psatdomain  LeftPortType=p1  RightPortType=p1  LConnTagsString=__newl0  RConnTagsString=__newr0  mask(Line){p3_4_5q=[100  230  60], p6q=80, p8q=[0.05], p9q=[0.001294461], p10q=[0.008941863e-6], p13_14_15q=[14.9 13.6 14.9], p16q=on}
      mask prompts: p3_4_5q "Power, Voltage and Frequency Ratings [MVA, kV, Hz]"; p6q "Length of line [km] (0 for p.u. parameters)"; p8q "Resistance [p.u. (Ohms/km)]"; p9q "Reactance [p.u. (H/km)]"; p10q "Susceptance [p.u. (F/km)]"; p13_14_15q "Imax, Pmax and Smax [p.u., p.u., p.u.]"; p16q "Connected"
      mask help: This block defines a pi model for a tree phase line.
      mask init:
      | [xp,yp] = fm_draw('pi');
      mask CallbackString: ||||||fm_block
      mask Display:
      | plot([-1  1  1 -1 -1],[-0.2 -0.2 0.2 0.2 -0.2])
      | color('blue')
      | plot(0.35*xp,0.2*yp)
  Line121 : PMComponent  Tag=PSATblock  Description=Power Flow  PhysicalDomain=psatdomain  LeftPortType=p1  RightPortType=p1  LConnTagsString=__newl0  RConnTagsString=__newr0  mask(Line){p3_4_5q=[532  230  60], p6q=224, p8q=[0.05], p9q=[0.001294461], p10q=[0.008941863e-6], p13_14_15q=[5.3 4.8 5.3], p16q=on}
      mask prompts: p3_4_5q "Power, Voltage and Frequency Ratings [MVA, kV, Hz]"; p6q "Length of line [km] (0 for p.u. parameters)"; p8q "Resistance [p.u. (Ohms/km)]"; p9q "Reactance [p.u. (H/km)]"; p10q "Susceptance [p.u. (F/km)]"; p13_14_15q "Imax, Pmax and Smax [p.u., p.u., p.u.]"; p16q "Connected"
      mask help: This block defines a pi model for a tree phase line.
      mask init:
      | [xp,yp] = fm_draw('pi');
      mask CallbackString: ||||||fm_block
      mask Display:
      | plot([-1  1  1 -1 -1],[-0.2 -0.2 0.2 0.2 -0.2])
      | color('blue')
      | plot(0.35*xp,0.2*yp)
  Line122 : PMComponent  Tag=PSATblock  Description=Power Flow  PhysicalDomain=psatdomain  LeftPortType=p1  RightPortType=p1  LConnTagsString=__newl0  RConnTagsString=__newr0  mask(Line){p3_4_5q=[100  230  60], p6q=80, p8q=[0.05], p9q=[0.001294461], p10q=[0.008941863e-6], p13_14_15q=[14.9 13.6 14.9], p16q=on}
      mask prompts: p3_4_5q "Power, Voltage and Frequency Ratings [MVA, kV, Hz]"; p6q "Length of line [km] (0 for p.u. parameters)"; p8q "Resistance [p.u. (Ohms/km)]"; p9q "Reactance [p.u. (H/km)]"; p10q "Susceptance [p.u. (F/km)]"; p13_14_15q "Imax, Pmax and Smax [p.u., p.u., p.u.]"; p16q "Connected"
      mask help: This block defines a pi model for a tree phase line.
      mask init:
      | [xp,yp] = fm_draw('pi');
      mask CallbackString: ||||||fm_block
      mask Display:
      | plot([-1  1  1 -1 -1],[-0.2 -0.2 0.2 0.2 -0.2])
      | color('blue')
      | plot(0.35*xp,0.2*yp)
  Line123 : PMComponent  Tag=PSATblock  Description=Power Flow  PhysicalDomain=psatdomain  LeftPortType=p1  RightPortType=p1  LConnTagsString=__newl0  RConnTagsString=__newr0  mask(Line){p3_4_5q=[100  400  60], p6q=38, p8q=[0.033806452], p9q=[0.000933966], p10q=[0.012626303e-6], p13_14_15q=[131.5 119.6 131.5], p16q=on}
      mask prompts: p3_4_5q "Power, Voltage and Frequency Ratings [MVA, kV, Hz]"; p6q "Length of line [km] (0 for p.u. parameters)"; p8q "Resistance [p.u. (Ohms/km)]"; p9q "Reactance [p.u. (H/km)]"; p10q "Susceptance [p.u. (F/km)]"; p13_14_15q "Imax, Pmax and Smax [p.u., p.u., p.u.]"; p16q "Connected"
      mask help: This block defines a pi model for a tree phase line.
      mask init:
      | [xp,yp] = fm_draw('pi');
      mask CallbackString: ||||||fm_block
      mask Display:
      | plot([-1  1  1 -1 -1],[-0.2 -0.2 0.2 0.2 -0.2])
      | color('blue')
      | plot(0.35*xp,0.2*yp)
  Line124 : PMComponent  Tag=PSATblock  Description=Power Flow  PhysicalDomain=psatdomain  LeftPortType=p1  RightPortType=p1  LConnTagsString=__newl0  RConnTagsString=__newr0  mask(Line){p3_4_5q=[100  138  60], p6q=6.2, p8q=[0.125], p9q=[0.000994719], p10q=[0.007460394e-6], p13_14_15q=[90.1 81.9 90.1], p16q=on}
      mask prompts: p3_4_5q "Power, Voltage and Frequency Ratings [MVA, kV, Hz]"; p6q "Length of line [km] (0 for p.u. parameters)"; p8q "Resistance [p.u. (Ohms/km)]"; p9q "Reactance [p.u. (H/km)]"; p10q "Susceptance [p.u. (F/km)]"; p13_14_15q "Imax, Pmax and Smax [p.u., p.u., p.u.]"; p16q "Connected"
      mask help: This block defines a pi model for a tree phase line.
      mask init:
      | [xp,yp] = fm_draw('pi');
      mask CallbackString: ||||||fm_block
      mask Display:
      | plot([-1  1  1 -1 -1],[-0.2 -0.2 0.2 0.2 -0.2])
      | color('blue')
      | plot(0.35*xp,0.2*yp)
  Line125 : PMComponent  Tag=PSATblock  Description=Power Flow  PhysicalDomain=psatdomain  LeftPortType=p1  RightPortType=p1  LConnTagsString=__newl0  RConnTagsString=__newr0  mask(Line){p3_4_5q=[100  230  60], p6q=9.8, p8q=[0.05], p9q=[0.001294461], p10q=[0.008941863e-6], p13_14_15q=[121.7 110.6 121.7], p16q=on}
      mask prompts: p3_4_5q "Power, Voltage and Frequency Ratings [MVA, kV, Hz]"; p6q "Length of line [km] (0 for p.u. parameters)"; p8q "Resistance [p.u. (Ohms/km)]"; p9q "Reactance [p.u. (H/km)]"; p10q "Susceptance [p.u. (F/km)]"; p13_14_15q "Imax, Pmax and Smax [p.u., p.u., p.u.]"; p16q "Connected"
      mask help: This block defines a pi model for a tree phase line.
      mask init:
      | [xp,yp] = fm_draw('pi');
      mask CallbackString: ||||||fm_block
      mask Display:
      | plot([-1  1  1 -1 -1],[-0.2 -0.2 0.2 0.2 -0.2])
      | color('blue')
      | plot(0.35*xp,0.2*yp)
  Line126 : PMComponent  Tag=PSATblock  Description=Power Flow  PhysicalDomain=psatdomain  LeftPortType=p1  RightPortType=p1  LConnTagsString=__newl0  RConnTagsString=__newr0  mask(Line){p3_4_5q=[100  230  60], p6q=6, p8q=[0.05], p9q=[0.001294461], p10q=[0.008941863e-6], p13_14_15q=[198.7 180.7 198.7], p16q=on}
      mask prompts: p3_4_5q "Power, Voltage and Frequency Ratings [MVA, kV, Hz]"; p6q "Length of line [km] (0 for p.u. parameters)"; p8q "Resistance [p.u. (Ohms/km)]"; p9q "Reactance [p.u. (H/km)]"; p10q "Susceptance [p.u. (F/km)]"; p13_14_15q "Imax, Pmax and Smax [p.u., p.u., p.u.]"; p16q "Connected"
      mask help: This block defines a pi model for a tree phase line.
      mask init:
      | [xp,yp] = fm_draw('pi');
      mask CallbackString: ||||||fm_block
      mask Display:
      | plot([-1  1  1 -1 -1],[-0.2 -0.2 0.2 0.2 -0.2])
      | color('blue')
      | plot(0.35*xp,0.2*yp)
  Line127 : PMComponent  Tag=PSATblock  Description=Power Flow  PhysicalDomain=psatdomain  LeftPortType=p1  RightPortType=p1  LConnTagsString=__newl0  RConnTagsString=__newr0  mask(Line){p3_4_5q=[100  230  60], p6q=16.1, p8q=[0.05], p9q=[0.001294461], p10q=[0.008941863e-6], p13_14_15q=[74.1 67.3 74.1], p16q=on}
      mask prompts: p3_4_5q "Power, Voltage and Frequency Ratings [MVA, kV, Hz]"; p6q "Length of line [km] (0 for p.u. parameters)"; p8q "Resistance [p.u. (Ohms/km)]"; p9q "Reactance [p.u. (H/km)]"; p10q "Susceptance [p.u. (F/km)]"; p13_14_15q "Imax, Pmax and Smax [p.u., p.u., p.u.]"; p16q "Connected"
      mask help: This block defines a pi model for a tree phase line.
      mask init:
      | [xp,yp] = fm_draw('pi');
      mask CallbackString: ||||||fm_block
      mask Display:
      | plot([-1  1  1 -1 -1],[-0.2 -0.2 0.2 0.2 -0.2])
      | color('blue')
      | plot(0.35*xp,0.2*yp)
  Line128 : PMComponent  Tag=PSATblock  Description=Power Flow  PhysicalDomain=psatdomain  LeftPortType=p1  RightPortType=p1  LConnTagsString=__newl0  RConnTagsString=__newr0  mask(Line){p3_4_5q=[100  138  60], p6q=6.2, p8q=[0.125], p9q=[0.000994719], p10q=[0.007460394e-6], p13_14_15q=[90.1 81.9 90.1], p16q=on}
      mask prompts: p3_4_5q "Power, Voltage and Frequency Ratings [MVA, kV, Hz]"; p6q "Length of line [km] (0 for p.u. parameters)"; p8q "Resistance [p.u. (Ohms/km)]"; p9q "Reactance [p.u. (H/km)]"; p10q "Susceptance [p.u. (F/km)]"; p13_14_15q "Imax, Pmax and Smax [p.u., p.u., p.u.]"; p16q "Connected"
      mask help: This block defines a pi model for a tree phase line.
      mask init:
      | [xp,yp] = fm_draw('pi');
      mask CallbackString: ||||||fm_block
      mask Display:
      | plot([-1  1  1 -1 -1],[-0.2 -0.2 0.2 0.2 -0.2])
      | color('blue')
      | plot(0.35*xp,0.2*yp)
  Line129 : PMComponent  Tag=PSATblock  Description=Power Flow  PhysicalDomain=psatdomain  LeftPortType=p1  RightPortType=p1  LConnTagsString=__newl0  RConnTagsString=__newr0  mask(Line){p3_4_5q=[100  230  60], p6q=9, p8q=[0.19253], p9q=[0.00021157], p10q=[0.416e-6], p13_14_15q=[810.6 736.9 810.6], p16q=on}
      mask prompts: p3_4_5q "Power, Voltage and Frequency Ratings [MVA, kV, Hz]"; p6q "Length of line [km] (0 for p.u. parameters)"; p8q "Resistance [p.u. (Ohms/km)]"; p9q "Reactance [p.u. (H/km)]"; p10q "Susceptance [p.u. (F/km)]"; p13_14_15q "Imax, Pmax and Smax [p.u., p.u., p.u.]"; p16q "Connected"
      mask help: This block defines a pi model for a tree phase cable.
      mask init:
      | [x,y] = fm_draw('circle');
      | [x1,y1] = fm_draw('semicircle');
      mask CallbackString: ||||||fm_block
      mask Display:
      | color('yellow')
      | plot(10+0.433*x,0.5+0.433*y)
      | plot(9.567+0.433*x,-0.25+0.433*y)
      | plot(10.433+0.433*x,-0.25+0.433*y)
      | color('black')
      | plot(-x1,y1)
      | plot(10+x,y,[0 10],[1 1],[0 10],[-1 -1])
  Line13 : PMComponent  Tag=PSATblock  Description=Power Flow  PhysicalDomain=psatdomain  LeftPortType=p1  RightPortType=p1  LConnTagsString=__newl0  RConnTagsString=__newr0  mask(Line){p3_4_5q=[100  400  60], p6q=169, p8q=[0.033806452], p9q=[0.000933966], p10q=[0.012626303e-6], p13_14_15q=[29.6 26.9 29.6], p16q=on}
      mask prompts: p3_4_5q "Power, Voltage and Frequency Ratings [MVA, kV, Hz]"; p6q "Length of line [km] (0 for p.u. parameters)"; p8q "Resistance [p.u. (Ohms/km)]"; p9q "Reactance [p.u. (H/km)]"; p10q "Susceptance [p.u. (F/km)]"; p13_14_15q "Imax, Pmax and Smax [p.u., p.u., p.u.]"; p16q "Connected"
      mask help: This block defines a pi model for a tree phase line.
      mask init:
      | [xp,yp] = fm_draw('pi');
      mask CallbackString: ||||||fm_block
      mask Display:
      | plot([-1  1  1 -1 -1],[-0.2 -0.2 0.2 0.2 -0.2])
      | color('blue')
      | plot(0.35*xp,0.2*yp)
  Line130 : PMComponent  Tag=PSATblock  Description=Power Flow  PhysicalDomain=psatdomain  LeftPortType=p1  RightPortType=p1  LConnTagsString=__newl0  RConnTagsString=__newr0  mask(Line){p3_4_5q=[100  138  60], p6q=4.3, p8q=[0.125], p9q=[0.000994719], p10q=[0.007460394e-6], p13_14_15q=[129.9 118.1 129.9], p16q=on}
      mask prompts: p3_4_5q "Power, Voltage and Frequency Ratings [MVA, kV, Hz]"; p6q "Length of line [km] (0 for p.u. parameters)"; p8q "Resistance [p.u. (Ohms/km)]"; p9q "Reactance [p.u. (H/km)]"; p10q "Susceptance [p.u. (F/km)]"; p13_14_15q "Imax, Pmax and Smax [p.u., p.u., p.u.]"; p16q "Connected"
      mask help: This block defines a pi model for a tree phase line.
      mask init:
      | [xp,yp] = fm_draw('pi');
      mask CallbackString: ||||||fm_block
      mask Display:
      | plot([-1  1  1 -1 -1],[-0.2 -0.2 0.2 0.2 -0.2])
      | color('blue')
      | plot(0.35*xp,0.2*yp)
  Line131 : PMComponent  Tag=PSATblock  Description=Power Flow  PhysicalDomain=psatdomain  LeftPortType=p1  RightPortType=p1  LConnTagsString=__newl0  RConnTagsString=__newr0  mask(Line){p3_4_5q=[100  230  60], p6q=12, p8q=[0.05], p9q=[0.001294461], p10q=[0.008941863e-6], p13_14_15q=[99.4 90.3 99.4], p16q=on}
      mask prompts: p3_4_5q "Power, Voltage and Frequency Ratings [MVA, kV, Hz]"; p6q "Length of line [km] (0 for p.u. parameters)"; p8q "Resistance [p.u. (Ohms/km)]"; p9q "Reactance [p.u. (H/km)]"; p10q "Susceptance [p.u. (F/km)]"; p13_14_15q "Imax, Pmax and Smax [p.u., p.u., p.u.]"; p16q "Connected"
      mask help: This block defines a pi model for a tree phase line.
      mask init:
      | [xp,yp] = fm_draw('pi');
      mask CallbackString: ||||||fm_block
      mask Display:
      | plot([-1  1  1 -1 -1],[-0.2 -0.2 0.2 0.2 -0.2])
      | color('blue')
      | plot(0.35*xp,0.2*yp)
  Line132 : PMComponent  Tag=PSATblock  Description=Power Flow  PhysicalDomain=psatdomain  LeftPortType=p1  RightPortType=p1  LConnTagsString=__newl0  RConnTagsString=__newr0  mask(Line){p3_4_5q=[100  138  60], p6q=12, p8q=[0.125], p9q=[0.000994719], p10q=[0.007460394e-6], p13_14_15q=[46.6 42.3 46.6], p16q=on}
      mask prompts: p3_4_5q "Power, Voltage and Frequency Ratings [MVA, kV, Hz]"; p6q "Length of line [km] (0 for p.u. parameters)"; p8q "Resistance [p.u. (Ohms/km)]"; p9q "Reactance [p.u. (H/km)]"; p10q "Susceptance [p.u. (F/km)]"; p13_14_15q "Imax, Pmax and Smax [p.u., p.u., p.u.]"; p16q "Connected"
      mask help: This block defines a pi model for a tree phase line.
      mask init:
      | [xp,yp] = fm_draw('pi');
      mask CallbackString: ||||||fm_block
      mask Display:
      | plot([-1  1  1 -1 -1],[-0.2 -0.2 0.2 0.2 -0.2])
      | color('blue')
      | plot(0.35*xp,0.2*yp)
  Line133 : PMComponent  Tag=PSATblock  Description=Power Flow  PhysicalDomain=psatdomain  LeftPortType=p1  RightPortType=p1  LConnTagsString=__newl0  RConnTagsString=__newr0  mask(Line){p3_4_5q=[100  230  60], p6q=9, p8q=[0.023], p9q=[0.00036046], p10q=[0.357e-6], p13_14_15q=[475.8 432.5 475.8], p16q=on}
      mask prompts: p3_4_5q "Power, Voltage and Frequency Ratings [MVA, kV, Hz]"; p6q "Length of line [km] (0 for p.u. parameters)"; p8q "Resistance [p.u. (Ohms/km)]"; p9q "Reactance [p.u. (H/km)]"; p10q "Susceptance [p.u. (F/km)]"; p13_14_15q "Imax, Pmax and Smax [p.u., p.u., p.u.]"; p16q "Connected"
      mask help: This block defines a pi model for a tree phase cable.
      mask init:
      | [x,y] = fm_draw('circle');
      | [x1,y1] = fm_draw('semicircle');
      mask CallbackString: ||||||fm_block
      mask Display:
      | color('yellow')
      | plot(10+0.433*x,0.5+0.433*y)
      | plot(9.567+0.433*x,-0.25+0.433*y)
      | plot(10.433+0.433*x,-0.25+0.433*y)
      | color('black')
      | plot(-x1,y1)
      | plot(10+x,y,[0 10],[1 1],[0 10],[-1 -1])
  Line134 : PMComponent  Tag=PSATblock  Description=Power Flow  PhysicalDomain=psatdomain  LeftPortType=p1  RightPortType=p1  LConnTagsString=__newl0  RConnTagsString=__newr0  mask(Line){p3_4_5q=[100  230  60], p6q=19, p8q=[0.05], p9q=[0.001294461], p10q=[0.008941863e-6], p13_14_15q=[62.8 57.1 62.8], p16q=on}
      mask prompts: p3_4_5q "Power, Voltage and Frequency Ratings [MVA, kV, Hz]"; p6q "Length of line [km] (0 for p.u. parameters)"; p8q "Resistance [p.u. (Ohms/km)]"; p9q "Reactance [p.u. (H/km)]"; p10q "Susceptance [p.u. (F/km)]"; p13_14_15q "Imax, Pmax and Smax [p.u., p.u., p.u.]"; p16q "Connected"
      mask help: This block defines a pi model for a tree phase line.
      mask init:
      | [xp,yp] = fm_draw('pi');
      mask CallbackString: ||||||fm_block
      mask Display:
      | plot([-1  1  1 -1 -1],[-0.2 -0.2 0.2 0.2 -0.2])
      | color('blue')
      | plot(0.35*xp,0.2*yp)
  Line135 : PMComponent  Tag=PSATblock  Description=Power Flow  PhysicalDomain=psatdomain  LeftPortType=p1  RightPortType=p1  LConnTagsString=__newl0  RConnTagsString=__newr0  mask(Line){p3_4_5q=[100  138  60], p6q=15.4, p8q=[0.125], p9q=[0.000994719], p10q=[0.007460394e-6], p13_14_15q=[36.3 33 36.3], p16q=on}
      mask prompts: p3_4_5q "Power, Voltage and Frequency Ratings [MVA, kV, Hz]"; p6q "Length of line [km] (0 for p.u. parameters)"; p8q "Resistance [p.u. (Ohms/km)]"; p9q "Reactance [p.u. (H/km)]"; p10q "Susceptance [p.u. (F/km)]"; p13_14_15q "Imax, Pmax and Smax [p.u., p.u., p.u.]"; p16q "Connected"
      mask help: This block defines a pi model for a tree phase line.
      mask init:
      | [xp,yp] = fm_draw('pi');
      mask CallbackString: ||||||fm_block
      mask Display:
      | plot([-1  1  1 -1 -1],[-0.2 -0.2 0.2 0.2 -0.2])
      | color('blue')
      | plot(0.35*xp,0.2*yp)
  Line136 : PMComponent  Tag=PSATblock  Description=Power Flow  PhysicalDomain=psatdomain  LeftPortType=p1  RightPortType=p1  LConnTagsString=__newl0  RConnTagsString=__newr0  mask(Line){p3_4_5q=[100  138  60], p6q=15.4, p8q=[0.125], p9q=[0.000994719], p10q=[0.007460394e-6], p13_14_15q=[36.3 33 36.3], p16q=on}
      mask prompts: p3_4_5q "Power, Voltage and Frequency Ratings [MVA, kV, Hz]"; p6q "Length of line [km] (0 for p.u. parameters)"; p8q "Resistance [p.u. (Ohms/km)]"; p9q "Reactance [p.u. (H/km)]"; p10q "Susceptance [p.u. (F/km)]"; p13_14_15q "Imax, Pmax and Smax [p.u., p.u., p.u.]"; p16q "Connected"
      mask help: This block defines a pi model for a tree phase line.
      mask init:
      | [xp,yp] = fm_draw('pi');
      mask CallbackString: ||||||fm_block
      mask Display:
      | plot([-1  1  1 -1 -1],[-0.2 -0.2 0.2 0.2 -0.2])
      | color('blue')
      | plot(0.35*xp,0.2*yp)
  Line137 : PMComponent  Tag=PSATblock  Description=Power Flow  PhysicalDomain=psatdomain  LeftPortType=p1  RightPortType=p1  LConnTagsString=__newl0  RConnTagsString=__newr0  mask(Line){p3_4_5q=[100  138  60], p6q=10.7, p8q=[0.125], p9q=[0.000994719], p10q=[0.007460394e-6], p13_14_15q=[52.2 47.5 52.2], p16q=on}
      mask prompts: p3_4_5q "Power, Voltage and Frequency Ratings [MVA, kV, Hz]"; p6q "Length of line [km] (0 for p.u. parameters)"; p8q "Resistance [p.u. (Ohms/km)]"; p9q "Reactance [p.u. (H/km)]"; p10q "Susceptance [p.u. (F/km)]"; p13_14_15q "Imax, Pmax and Smax [p.u., p.u., p.u.]"; p16q "Connected"
      mask help: This block defines a pi model for a tree phase line.
      mask init:
      | [xp,yp] = fm_draw('pi');
      mask CallbackString: ||||||fm_block
      mask Display:
      | plot([-1  1  1 -1 -1],[-0.2 -0.2 0.2 0.2 -0.2])
      | color('blue')
      | plot(0.35*xp,0.2*yp)
  Line138 : PMComponent  Tag=PSATblock  Description=Power Flow  PhysicalDomain=psatdomain  LeftPortType=p1  RightPortType=p1  LConnTagsString=__newl0  RConnTagsString=__newr0  mask(Line){p3_4_5q=[100  230  60], p6q=124, p8q=[0.05], p9q=[0.001294461], p10q=[0.008941863e-6], p13_14_15q=[9.6 8.7 9.6], p16q=on}
      mask prompts: p3_4_5q "Power, Voltage and Frequency Ratings [MVA, kV, Hz]"; p6q "Length of line [km] (0 for p.u. parameters)"; p8q "Resistance [p.u. (Ohms/km)]"; p9q "Reactance [p.u. (H/km)]"; p10q "Susceptance [p.u. (F/km)]"; p13_14_15q "Imax, Pmax and Smax [p.u., p.u., p.u.]"; p16q "Connected"
      mask help: This block defines a pi model for a tree phase line.
      mask init:
      | [xp,yp] = fm_draw('pi');
      mask CallbackString: ||||||fm_block
      mask Display:
      | plot([-1  1  1 -1 -1],[-0.2 -0.2 0.2 0.2 -0.2])
      | color('blue')
      | plot(0.35*xp,0.2*yp)
